simulink model "LDPC_sim"  (R2024a)
(part 16 of 20)

true;true;true;true;true;true;true;true;true;true;true;true;true;true;true;true;true;true;true;true;true;true;true;true;true;true;true;true;true;true;true;true;true;true;true;true;true;true;true;true;true;true;true;true;true;true;true;true;true;true;true;true;true;true;true;true;true;true;true;true;true;true;true;true;true;true;true;true;true;true;true;true;true;true;true;true;true;true;true;true;true;true;true;true;true;true;true;true;true;true;true;true;true;true;true;true;true;true;true;true;true;true;true;true;true;true;true;true;true;true;true;true;true;true;true;true;true;true;true;true;true;true;true;true;true;true;true;true;true;true;true;true;true;true;true;true;true;true;true;true;true;true;true;true;true;true;true;true;true;true;true;true;true;true;true;true;true;true;true;true;true;true;true;true;true;true;true;true;true;true;true;true;true;true;true;true;true;true;true;true;true;true;true;true;true;true;true;true;true;true;true;true;true;true;true;true;true;true;true;true;true;true;true;true;true;true;true;true;true;true;true;true;true;true;true;true;true;true;true;true;true;true;true;true;true;true;true;true;true;true;true;true;true;true;true;true;true;true;true;true;true;true;true;true;true;true;true;true;true;true;true;true;true;true;true;true;true;true;true;true;true;true;true;true;true;true;true;true;true;true;true;true;true;true;true;true;true;true;true;true;true;true;true;true;true;true;true;true;true;true;true;true;true;true;true;true;true;true;true;true;true;true;true;true;true;true;true;true;true;true;true;true;true;true;true;true;true;true;true;true;true;true;true;true;true;true;true;true;true;true;true;true;true;true;true;true;true;true;true;true;true;true;true;true;true;true;true;true;true;true;true;true;true;true;true;true;true;true;true;true;true;true;true;true;true;true;true;true;true;true;true;true;true;true;true;true;true;true;true;true;true;true;true;true;true;true;true;true;true;true;true;true;true;true;true;true;true;true;true;true;true;true;true;true;true;true;true;true;true;true;true;true;true;true;true;true;true;true;true;true;true;true;true;true;true;true;true;true;true;true;true;true;true;true;true;true;true;true;true;true;true;true;true;true;true;true;true;true;true;true;true;true;true;true;true;true;true;true;true;true;true;true;true;true;true;true;true;true;true;true;true;true;true;true;true;true;true;true;true;true;true;true;true;true;true;true;true;true;true;true;true;true;true;true;true;true;true;true;true;true;true;true;true;true;true;true;true;true;true;true;true;true;true;true;true;true;true;true;true;true;true;true;true;true;true;true;true;true;true;true;true;true;true;true;true;true;true;true;true;true;true;true;true;true;true;true;true;true;true;true;true;true;true;true;true;true;true;true;true;true;true;true;true;true;true;true;true;true;true;true;true;true;true;true;true;true;true;true;true;true;true;true;true;true;true;true;true;true;true;true;true;true;true;true;true;true;true;true;true;true;true;true;true;true;true;true;true;true;true;true;true;true;true;true;true;true;true;true;true;true;true;true;true;true;true;true;true;true;true;true;true;true;true;true;true;true;true;true;true;true;true;true;true;true;true;true;true;true;true;true;true;true;true;true;true;true;true;true;true;true;true;true;true;true;true;true;true;true;true;true;true;true;true;true;true;true;true;true;true;true;true;true;true;true;true;true;true;true;true;true;true;true;true;true;true;true;true;true;true;true;true;true;true;true;true;true;true;true;true;true;true;true;true;true;true;true;true;true;true;true;true;true;true;true;true;true;true;true;true;true;true;true;true;true;true;true;true;true;true;true;true;true;true;true;true;true;true;true;true;true;true;true;true;true;true;true;true;true;true;true;true;true;true;true;true;true;true;true;true;true;true;true;true;true;true;true;true;true;true;true;true;true;true;true;true;true;true;true;true;true;true;true;true;true;true;true;true;true;true;true;true;true;true;true;true;true;true;true;true;true;true;true;true;true;true;true;true;true;true;true;true;true;true;true;true;true;true;true;true;true;true;true;true;true;true;true;true;true;true;true;true;true;true;true;true;true;true;true;true;true;true;true;true;true;true;true;true;true;true;true;true;true;true;true;true;true;true;true;true;true;true;true;true;true;true;true;true;true;true;true;true;true;true;true;true;true;true;true;true;true;true;true;true;true;true;true;true;true;true;true;true;true;true;true;true;true;true;true;true;true;true;true;true;true;true;true;true;true;true;true;true;true;true;true;true;true;true;true;true;true;true;true;true;true;true;true;true;true;true;true;true;true;true;true;true;true;true;true;true;true;true;true;true;true;true;true;true;true;true;true;true;true;true;true;true;true;true;true;true;true;true;true;true;true;true;true;true;true;true;true;true;true;true;true;true;true;true;true;true;true;true;true;true;true;true;true;true;true;true;true;true;true;true;true;true;true;true;true;true;true;true;true;true;true;true;true;true;true;true;true;true;true;true;true;true;true;true;true;true;true;true;true;true;true;true;true;true;true;true;true;true;true;true;true;true;true;true;true;true;true;true;true;true;true;true;true;true;true;true;true;true;true;true;true;true;true;true;true;true;true;true;true;true;true;true;true;true;true;true;true;true;true;true;true;true;true;true;true;true;true;true;true;true;true;true;true;true;true;true;true;true;true;true;true;true;true;true;true;true;true;true;true;true;true;true;true;true;true;true;true;true;true;true;true;true;true;true;true;true;true;true;true;true;true;true;true;true;true;true;true;true;true;true;true;true;true;true;true;true;true;true;true;true;true;true;true;true;true;true;true;true;true;true;true;true;true;true;true;true;true;true;true;true;true;true;true;true;true;true;true;true;true;true;true;true;true;true;true;true;true;true;true;true;true;true;true;true;true;true;true;true;true;true;true;true;true;true;true;true;true;true;true;true;true;true;true;true;true;true;true;true;true;true;true;true;true;true;true;true;true;true;true;true;true;true;true;true;true;true;true;true;true;true;true;true;true;true;true;true;true;true;true;true;true;true;true;true;true;true;true;true;true;true;true;true;true;true;true;true;true;true;true;true;true;true;true;true;true;true;true;true;true;true;true;true;true;true;true;true;true;true;true;true;true;true;true;true;true;true;true;true;true;true;true;true;true;true;true;true;true;true;true;true;true;true;true;true;true;true;true;true;true;true;true;true;true;true;true;true;true;true;true;true;true;true;true;true;true;true;true;true;true;true;true;true;true;true;true;true;true;true;true;true;true;true;true;true;true;true;true;true;true;true;true;true;true;true;true;true;true;true;true;true;true;true;true;true;true;true;true;true;true;true;true;true;true;true;true;true;true;true;true;true;true;true;true;true;true;true;true;true;true;true;true;true;true;true;true;true;true;true;true;true;true;true;true;true;true;true;true;true;true;true;true;true;true;true;true;true;true;true;true;true;true;true;true;true;true;true;true;true;true;true;true;true;true;true;true;true;true;true;true;true;true;true;true;true;true;true;true;true;true;true;true;true;true;true;true;true;true;true;true;true;true;true;true;true;true;true;true;true;true;true;true;true;true;true;true;true;true;true;true;true;true;true;true;true;true;true;true;true;true;true;true;true;true;true;true;true;true;true;true;true;true;true;true;true;true;true;true;true;true;true;true;true;true;true;true;true;true;true;true;true;true;true;true;true;true;true;true;true;true;true;true;true;true;true;true;true;true;true;true;true;true;true;true;true;true;true;true;true;true;true;true;true;true;true;true;true;true;true;true;true;true;true;true;true;true;true;true;true;true;true;true;true;true;true;true;true;true;true;true;true;true;true;true;true;true;true;true;true;true;true;true;true;true;true;true;true;true;true;true;true;true;true;true;true;true;true;true;true;true;true;true;true;true;true;true;true;true;true;true;true;true;true;true;true;true;true;true;true;true;true;true;true;true;true;true;true;true;true;true;true;true;true;true;true;true;true;true;true;true;true;true;true;true;true;true;true;true;true;true;true;true;true;true;true;true;true;true;true;true;true;true;true;true;true;true;true;true;true;true;true;true;true;true;true;true;true;true;true;true;true;true;true;true;true;true;true;true;true;true;true;true;true;true;true;true;true;true;true;true;true;true;true;true;true;true;true;true;true;true;true;true;true;true;true;true;true;true;true;true;true;true;true;true;true;true;true;true;true;true;true;true;true;true;true;true;true;true;true;true;true;true;true;true;true;true;true;true;true;true;true;true;true;true;true;true;true;true;true;true;true;true;true;true;true;true;true;true;true;true;true;true;true;true;true;true;true;true;true;true;true;true;true;true;true;true;true;true;true;true;true;true;true;true;true;true;true;true;true;true;true;true;true;true;true;true;true;true;true;true;true;true;true;true;true;true;true;true;true;true;true;true;true;true;true;true;true;true;true;true;true;true;true;true;true;true;true;true;true;true;true;true;true;true;true;true;true;true;true;true;true;true;true;true;true;true;true;true;true;true;true;true;true;true;true;true;true;true;true;true;true;true;true;true;true;true;true;true;true;true;true;true;true;true;true;true;true;true;true;true;true;true;true;true;true;true;true;true;true;true;true;true;true;true;true;true;true;true;true;true;true;true;true;true;true;true;true;true;true;true;true;true;true;true;true;true;true;true;true;true;true;true;true;true;true;true;true;true;true;true;true;true;true;true;true;true;true;true;true;true;true;true;true;true;true;true;true;true;true;true;true;true;true;true;true;true;true;true;true;true;true;true;true;true;true;true;true;true;true;true;true;true;true;true;true;true;true;true;true;true;true;true;true;true;true;true;true;true;true;true;true;true;true;true;true;true;true;true;true;true;true;true;true;true;true;true;true;true;true;true;true;true;true;true;true;true;true;true;true;true;true;true;true;true;true;true;true;true;true;true;true;true;true;true;true;true;true;true;true;true;true;true;true;true;true;true;true;true;true;true;true;true;true;true;true;true;true;true;true;true;true;true;true;true;true;true;true;true;true;true;true;true;true;true;true;true;true;true;true;true;true;true;true;true;true;true;true;true;true;true;true;true;true;true;true;true;true;true;true;true;true;true;true;true;true;true;true;true;true;true;true;true;true;true;true;true;true;true;true;true;true;true;true;true;true;true;true;true;true;true;true;true;true;true;true;true;true;true;true;true;true;true;true;true;true;true;true;true;true;true;true;true;true;true;true;true;true;true;true;true;true;true;true;true;true;true;true;true;true;true;true;true;true;true;true;true;true;true;true;true;true;true;true;true;true;true;true;true;true;true;true;true;true;true;true;true;true;true;true;true;true;true;true;true;true;true;true;true;true;true;true;true;true;true;true;true;true;true;true;true;true;true;true;true;true;true;true;true;true;true;true;true;true;true;true;true;true;true;true;true;true;true;true;true;true;true;true;true;true;true;true;true;true;true;true;true;true;true;true;true;true;true;true;true;true;true;true;true;true;true;true;true;true;true;true;true;true;true;true;true;true;true;true;true;true;true;true;true;true;true;true;true;true;true;true;true;true;true;true;true;true;true;true;true;true;true;true;true;true;true;true;true;true;true;true;true;true;true;true;true;true;true;true;true;true;true;true;true;true;true;true;true;true;true;true;true;true;true;true;true;true;true;true;true;true;true;true;true;true;true;true;true;true;true;true;true;true;true;true;true;true;true;true;true;true;true;true;true;true;true;true;true;true;true;true;true;true;true;true;true;true;true;true;true;true;true;true;true;true;true;true;true;true;true;true;true;true;true;true;true;true;true;true;true;true;true;true;true;true;true;true;true;true;true;true;true;true;true;true;true;true;true;true;true;true;true;true;true;true;true;true;true;true;true;true;true;true;true;true;true;true;true;true;true;true;true;true;true;true;true;true;true;true;true;true;true;true;true;true;true;true;true;true;true;true;true;true;true;true;true;true;true;true;true;true;true;true;true;true;true;true;true;true;true;true;true;true;true;true;true;true;true;true;true;true;true;true;true;true;true;true;true;true;true;true;true;true;true;true;true;true;true;true;true;true;true;true;true;true;true;true;true;true;true;true;true;true;true;true;true;true;true;true;true;true;true;true;true;true;true;true;true;true;true;true;true;true;true;true;true;true;true;true;true;true;true;true;true;true;true;true;true;true;true;true;true;true;true;true;true;true;true;true;true;true;true;true;true;true;true;true;true;true;true;true;true;true;true;true;true;true;true;true;true;true;true;true;true;true;true;true;true;true;true;true;true;true;true;true;true;true;true;true;true;true;true;true;true;true;true;true;true;true;true;true;true;true;true;true;true;true;true;true;true;true;true;true;true;true;true;true;true;true;true;true;true;true;true;true;true;true;true;true;true;true;true;true;true;true;true;true;true;true;true;true;true;true;true;true;true;true;true;true;true;true;true;true;true;true;true;true;true;true;true;true;true;true;true;true;true;true;true;true;true;true;true;true;true;true;true;true;true;true;true;true;true;true;true;true;true;true;true;true;true;true;true;true;true;true;true;true;true;true;true;true;true;true;true;true;true;true;true;true;true;true;true;true;true;true;true;true;true;true;true;true;true;true;true;true;true;true;true;true;true;true;true;true;true;true;true;true;true;true;true;true;true;true;true;true;true;true;true;true;true;true;true;true;true;true;true;true;true;true;true;true;true;true;true;true;true;true;true;true;true;true;true;true;true;true;true;true;true;true;true;true;true;true;true;true;true;true;true;true;true;true;true;true;true;true;true;true;true;true;true;true;true;true;true;true;true;true;true;true;true;true;true;true;true;true;true;true;true;true;true;true;true;true;true;true;true;true;true;true;true;true;true;true;true;true;true;true;true;true;true;true;true;true;true;true;true;true;true;true;true;true;true;true;true;true;true;true;true;true;true;true;true;true;true;true;true;true;true;true;true;true;true;true;true;true;true;true;true;true;true;true;true;true;true;true;true;true;true;true;true;true;true;true;true;true;true;true;true;true;true;true;true;true;true;true;true;true;true;true;true;true;true;true;true;true;true;true;true;true;true;true;true;true;true;true;true;true;true;true;true;true;true;true;true;true;true;true;true;true;true;true;true;true;true;true;true;true;true;true;true;true;true;true;true;true;true;true;true;true;true;true;true;true;true;true;true;true;true;true;true;true;true;true;true;true;true;true;true;true;true;true;true;true;true;true;true;true;true;true;true;true;true;true;true;true;true;true;true;true;true;true;true;true;true;true;true;true;true;true;true;true;true;true;true;true;true;true;true;true;true;true;true;true;true;true;true;true;true;true;true;true;true;true;true;true;true;true;true;true;true;true;true;true;true;true;true;true;true;true;true;true;true;true;true;true;true;true;true;true;true;true;true;true;true;true;true;true;true;true;true;true;true;true;true;true;true;true;true;true;true;true;true;true;true;true;true;true;true;true;true;true;true;true;true;true;true;true;true;true;true;true;true;true;true;true;true;true;true;true;true;true;true;true;true;true;true;true;true;true;true;true;true;true;true;true;true;true;true;true;true;true;true;true;true;true;true;true;true;true;true;true;true;true;true;true;true;true;true;true;true;true;true;true;true;true;true;true;true;true;true;true;true;true;true;true;true;true;true;true;true;true;true;true;true;true;true;true;true;true;true;true;true;true;true;true;true;true;true;true;true;true;true;true;true;true;true;true;true;true;true;true;true;true;true;true;true;true;true;true;true;true;true;true;true;true;true;true;true;true;true;true;true;true;true;true;true;true;true;true;true;true;true;true;true;true;true;true;true;true;true;true;true;true;true;true;true;true;true;true;true;true;true;true;true;true;true;true;true;true;true;true;true;true;true;true;true;true;true;true;true;true;true;true;true;true;true;true;true;true;true;true;true;true;true;true;true;true;true;true;true;true;true;true;true;true;true;true;true;true;true;true;true;true;true;true;true;true;true;true;true;true;true;true;true;true;true;true;true;true;true;true;true;true;true;true;true;true;true;true;true;true;true;true;true;true;true;true;true;true;true;true;true;true;true;true;true;true;true;true;true;true;true;true;true;true;true;true;true;true;true;true;true;true;true;true;true;true;true;true;true;true;true;true;true;true;true;true;true;true;true;true;true;true;true;true;true;true;true;true;true;true;true;true;true;true;true;true;true;true;true;true;true;true;true;true;true;true;true;true;true;true;true;true;true;true;true;true;true;true;true;true;true;true;true;true;true;true;true;true;true;true;true;true;true;true;true;true;true;true;true;true;true;true;true;true;true;true;true;true;true;true;true;true;true;true;true;true;true;true;true;true;true;true;true;true;true;true;true;true;true;true;true;true;true;true;true;true;true;true;true;true;true;true;true;true;true;true;true;true;true;true;true;true;true;true;true;true;true;true;true;true;true;true;true;true;true;true;true;true;true;true;true;true;true;true;true;true;true;true;true;true;true;true;true;true;true;true;true;true;true;true;true;true;true;true;true;true;true;true;true;true;true;true;true;true;true;true;true;true;true;true;true;true;true;true;true;true;true;true;true;true;true;true;true;true;true;true;true;true;true;true;true;true;true;true;true;true;true;true;true;true;true;true;true;true;true;true;true;true;true;true;true;true;true;true;true;true;true;true;true;true;true;true;true;true;true;true;true;true;true;true;true;true;true;true;true;true;true;true;true;true;true;true;true;true;true;true;true;true;true;true;true;true;true;true;true;true;true;true;true;true;true;true;true;true;true;true;true;true;true;true;true;true;true;true;true;true;true;true;true;true;true;true;true;true;true;true;true;true;true;true;true;true;true;true;true;true;true;true;true;true;true;true;true;true;true;true;true;true;true;true;true;true;true;true;true;true;true;true;true;true;true;true;true;true;true;true;true;true;true;true;true;true;true;true;true;true;true;true;true;true;true;true;true;true;true;true;true;true;true;true;true;true;true;true;true;true;true;true;true;true;true;true;true;true;true;true;true;true;true;true;true;true;true;true;true;true;true;true;true;true;true;true;true;true;true;true;true;true;true;true;true;true;true;true;true;true;true;true;true;true;true;true;true;true;true;true;true;true;true;true;true;true;true;true;true;true;true;true;true;true;true;true;true;true;true;true;true;true;true;true;true;true;true;true;true;true;true;true;true;true;true;true;true;true;true;true;true;true;true;true;true;true;true;true;true;true;true;true;true;true;true;true;true;true;true;true;true;true;true;true;true;true;true;true;true;true;true;true;true;true;true;true;true;true;true;true;true;true;true;true;true;true;true;true;true;true;true;true;true;true;true;true;true;true;true;true;true;true;true;true;true;true;true;true;true;true;true;true;true;true;true;true;true;true;true;true;true;true;true;true;true;true;true;true;true;true;true;true;true;true;true;true;true;true;true;true;true;true;true;true;true;true;true;true;true;true;true;true;true;true;true;true;true;true;true;true;true;true;true;true;true;true;true;true;true;true;true;true;true;true;true;true;true;true;true;true;true;true;true;true;true;true;true;true;true;true;true;true;true;true;true;true;true;true;true;true;true;true;true;true;true;true;true;true;true;true;true;true;true;true;true;true;true;true;true;true;true;true;true;true;true;true;true;true;true;true;true;true;true;true;true;true;true;true;true;true;true;true;true;true;true;true;true;true;true;true;true;true;true;true;true;true;true;true;true;true;true;true;true;true;true;true;true;true;true;true;true;true;true;true;true;true;true;true;true;true;true;true;true;true;true;true;true;true;true;true;true;true;true;true;true;true;true;true;true;true;true;true;true;true;true;true;true;true;true;true;true;true;true;true;true;true;true;true;true;true;true;true;true;true;true;true;true;true;true;true;true;true;true;true;true;true;true;true;true;true;true;true;true;true;true;true;true;true;true;true;true;true;true;true;true;true;true;true;true;true;true;true;true;true;true;true;true;true;true;true;true;true;true;true;true;true;true;true;true;true;true;true;true;true;true;true;true;true;true;true;true;true;true;true;true;true;true;true;true;true;true;true;true;true;true;true;true;true;true;true;true;true;true;true;true;true;true;true;true;true;true;true;true;true;true;true;true;true;true;true;true;true;true;true;true;true;true;true;true;true;true;true;true;true;true;true;true;true;true;true;true;true;true;true;true;true;true;true;true;true;true;true;true;true;true;true;true;true;true;true;true;true;true;true;true;true;true;true;true;true;true;true;true;true;true;true;true;true;true;true;true;true;true;true;true;true;true;true;true;true;true;true;true;true;true;true;true;true;true;true;true;true;true;true;true;true;true;true;true;true;true;true;true;true;true;true;true;true;true;true;true;true;true;true;true;true;true;true;true;true;true;true;true;true;true;true;true;true;true;true;true;true;true;true;true;true;true;true;true;true;true;true;true;true;true;true;true;true;true;true;true;true;true;true;true;true;true;true;true;true;true;true;true;true;true;true;true;true;true;true;true;true;true;true;true;true;true;true;true;true;true;true;true;true;true;true;true;true;true;true;true;true;true;true;true;true;true;true;true;true;true;true;true;true;true;true;true;true;true;true;true;true;true;true;true;true;true;true;true;true;true;true;true;true;true;true;true;true;true;true;true;true;true;true;true;true;true;true;true;true;true;true;true;true;true;true;true;true;true;true;true;true;true;true;true;true;true;true;true;true;true;true;true;true;true;true;true;true;true;true;true;true;true;true;true;true;true;true;true;true;true;true;true;true;true;true;true;true;true;true;true;true;true;true;true;true;true;true;true;true;true;true;true;true;true;true;true;true;true;true;true;true;true;true;true;true;true;true;true;true;true;true;true;true;true;true;true;true;true;true;true;true;true;true;true;true;true;true;true;true;true;true;true;true;true;true;true;true;true;true;true;true;true;true;true;true;true;true;true;true;true;true;true;true;true;true;true;true;true;true;true;true;true;true;true;true;true;true;true;true;true;true;true;true;true;true;true;true;true;true;true;true;true;true;true;true;true;true;true;true;true;true;true;true;true;true;true;true;true;true;true;true;true;true;true;true;true;true;true;true;true;true;true;true;true;true;true;true;true;true;true;true;true;true;true;true;true;true;true;true;true;true;true;true;true;true;true;true;true;true;true;true;true;true;true;true;true;true;true;true;true;true;true;true;true;true;true;true;true;true;true;true;true;true;true;true;true;true;true;true;true;true;true;true;true;true;true;true;true;true;true;true;true;true;true;true;true;true;true;true;true;true;true;true;true;true;true;true;true;true;true;true;true;true;true;true;true;true;true;true;true;true;true;true;true;true;true;true;true;true;true;true;true;true;true;true;true;true;true;true;true;true;true;true;true;true;true;true;true;true;true;true;true;true;true;true;true;true;true;true;true;true;true;true;true;true;true;true;true;true;true;true;true;true;true;true;true;true;true;true;true;true;true;true;true;true;true;true;true;true;true;true;true;true;true;true;true;true;true;true;true;true;true;true;true;true;true;true;true;true;true;true;true;true;true;true;true;true;true;true;true;true;true;true;true;true;true;true;true;true;true;true;true;true;true;true;true;true;true;true;true;true;true;true;true;true;true;true;true;true;true;true;true;true;true;true;true;true;true;true;true;true;true;true;true;true;true;true;true;true;true;true;true;true;true;true;true;true;true;true;true;true;true;true;true;true;true;true;true;true;true;true;true;true;true;true;true;true;true;true;true;true;true;true;true;true;true;true;true;true;true;true;true;true;true;true;true;true;true;true;true;true;true;true;true;true;true;true;true;true;true;true;true;true;true;true;true;true;true;true;true;true;true;true;true;true;true;true;true;true;true;true;true;true;true;true;true;true;true;true;true;true;true;true;true;true;true;true;true;true;true;true;true;true;true;true;true;true;true;true;true;true;true;true;true;true;true;true;true;true;true;true;true;true;true;true;true;true;true;true;true;true;true;true;true;true;true;true;true;true;true;true;true;true;true;true;true;true;true;true;true;true;true;true;true;true;true;true;true;true;true;true;true;true;true;true;true;true;true;true;true;true;true;true;true;true;true;true;true;true;true;true;true;true;true;true;true;true;true;true;true;true;true;true;true;true;true;true;true;true;true;true;true;true;true;true;true;true;true;true;true;true;true;true;true;true;true;true;true;true;true;true;true;true;true;true;true;true;true;true;true;true;true;true;true;true;true;true;true;true;true;true;true;true;true;true;true;true;true;true;true;true;true;true;true;true;true;true;true;true;true;true;true;true;true;true;true;true;true;true;true;true;true;true;true;true;true;true;true;true;true;true;true;true;true;true;true;true;true;true;true;true;true;true;true;true;true;true;true;true;true;true;true;true;true;true;true;true;true;true;true;true;true;true;true;true;true;true;true;true;true;true;true;true;true;true;true;true;true;true;true;true;true;true;true;true;true;true;true;true;true;true;true;true;true;true;true;true;true;true;true;true;true;true;true;true;true;true;true;true;true;true;true;true;true;true;true;true;true;true;true;true;true;true;true;true;true;true;true;true;true;true;true;true;true;true;true;true;true;true;true;true;true;true;true;true;true;true;true;true;true;true;true;true;true;true;true;true;true;true;true;true;true;true;true;true;true;true;true;true;true;true;true;true;true;true;true;true;true;true;true;true;true;true;true;true;true;true;true;true;true;true;true;true;true;true;true;true;true;true;true;true;true;true;true;true;true;true;true;true;true;true;true;true;true;true;true;true;true;true;true;true;true;true;true;true;true;true;true;true;true;true;true;true;true;true;true;true;true;true;true;true;true;true;true;true;true;true;true;true;true;true;true;true;true;true;true;true;true;true;true;true;true;true;true;true;true;true;true;true;true;true;true;true;true;true;true;true;true;true;true;true;true;true;true;true;true;true;true;true;true;true;true;true;true;true;true;true;true;true;true;true;true;true;true;true;true;true;true;true;true;true;true;true;true;true;true;true;true;true;true;true;true;true;true;true;true;true;true;true;true;true;true;true;true;true;true;true;true;true;true;true;true;true;true;true;true;true;true;true;true;true;true;true;true;true;true;true;true;true;true;true;true;true;true;true;true;true;true;true;true;true;true;true;true;true;true;true;true;true;true;true;true;true;true;true;true;true;true;true;true;true;true;true;true;true;true;true;true;true;true;true;true;true;true;true;true;true;true;true;true;true;true;true;true;true;true;true;true;true;true;true;true;true;true;true;true;true;true;true;true;true;true;true;true;true;true;true;true;true;true;true;true;true;true;true;true;true;true;true;true;true;true;true;true;true;true;true;true;true;true;true;true;true;true;true;true;true;true;true;true;true;true;true;true;true;true;true;true;true;true;true;true;true;true;true;true;true;true;true;true;true;true;true;true;true;true;true;true;true;true;true;true;true;true;true;true;true;true;true;true;true;true;true;true;true;true;true;true;true;true;true;true;true;true;true;true;true;true;true;true;true;true;true;true;true;true;true;true;true;true;true;true;true;true;true;true;true;true;true;true;true;true;true;true;true;true;true;true;true;true;true;true;true;true;true;true;true;true;true;true;true;true;true;true;true;true;true;true;true;true;true;true;true;true;true;true;true;true;true;true;true;true;true;true;true;true;true;true;true;true;true;true;true;true;true;true;true;true;true;true;true;true;true;true;true;true;true;true;true;true;true;true;true;true;true;true;true;true;true;true;true;true;true;true;true;true;true;true;true;true;true;true;true;true;true;true;true;true;true;true;true;true;true;true;true;true;true;true;true;true;true;true;true;true;true;true;true;true;true;true;true;true;true;true;true;true;true;true;true;true;true;true;true;true;true;true;true;true;true;true;true;true;true;true;true;true;true;true;true;true;true;true;true;true;true;true;true;true;true;true;true;true;true;true;true;true;true;true;true;true;true;true;true;true;true;true;true;true;true;true;true;true;true;true;true;true;true;true;true;true;true;true;true;true;true;true;true;true;true;true;true;true;true;true;true;true;true;true;true;true;true;true;true;true;true;true;true;true;true;true;true;true;true;true;true;true;true;true;true;true;true;true;true;true;true;true;true;true;true;true;true;true;true;true;true;true;true;true;true;true;true;true;true;true;true;true;true;true;true;true;true;true;true;true;true;true;true;true;true;true;true;true;true;true;true;true;true;true;true;true;true;true;true;true;true;true;true;true;true;true;true;true;true;true;true;true;true;true;true;true;true;true;true;true;true;true;true;true;true;true;true;true;true;true;true;true;true;true;true;true;true;true;true;true;true;true;true;true;true;true;true;true;true;true;true;true;true;true;true;true;true;true;true;true;true;true;true;true;true;true;true;true;true;true;true;true;true;true;true;true;true;true;true;true;true;true;true;true;true;true;true;true;true;true;true;true;true;true;true;true;true;true;true;true;true;true;true;true;true;true;true;true;true;true;true;true;true;true;true;true;true;true;true;true;true;true;true;true;true;true;true;true;true;true;true;true;true;true;true;true;true;true;true;true;true;true;true;true;true;true;true;true;true;true;true;true;true;true;true;true;true;true;true;true;true;true;true;true;true;true;true;true;true;true;true;true;true;true;true;true;true;true;true;true;true;true;true;true;true;true;true;true;true;true;true;true;true;true;true;true;true;true;true;true;true;true;true;true;true;true;true;true;true;true;true;true;true;true;true;true;true;true;true;true;true;true;true;true;true;true;true;true;true;true;true;true;true;true;true;true;true;true;true;true;true;true;true;true;true;true;true;true;true;true;true;true;true;true;true;true;true;true;true;true;true;true;true;true;true;true;true;true;true;true;true;true;true;true;true;true;true;true;true;true;true;true;true;true;true;true;true;true;true;true;true;true;true;true;true;true;true;true;true;true;true;true;true;true;true;true;true;true;true;true;true;true;true;true;true;true;true;true;true;true;true;true;true;true;true;true;true;true;true;true;true;true;true;true;true;true;true;true;true;true;true;true;true;true;true;true;true;true;true;true;true;true;true;true;true;true;true;true;true;true;true;true;true;true;true;true;true;true;true;true;true;true;true;true;true;true;true;true;true;true;true;true;true;true;true;true;true;true;true;true;true;true;true;true;true;true;true;true;true;true;true;true;true;true;true;true;true;true;true;true;true;true;true;true;true;true;true;true;true;true;true;true;true;true;true;true;true;true;true;true;true;true;true;true;true;true;true;true;true;true;true;true;true;true;true;true;true;true;true;true;true;true;true;true;true;true;true;true;true;true;true;true;true;true;true;true;true;true;true;true;true;true;true;true;true;true;true;true;true;true;true;true;true;true;true;true;true;true;true;true;true;true;true;true;true;true;true;true;true;true;true;true;true;true;true;true;true;true;true;true;true;true;true;true;true;true;true;true;true;true;true;true;true;true;true;true;true;true;true;true;true;true;true;true;true;true;true;true;true;true;true;true;true;true;true;true;true;true;true;true;true;true;true;true;true;true;true;true;true;true;true;true;true;true;true;true;true;true;true;true;true;true;true;true;true;true;true;true;true;true;true;true;true;true;true;true;true;true;true;true;true;true;true;true;true;true;true;true;true;true;true;true;true;true;true;true;true;true;true;true;true;true;true;true;true;true;true;true;true;true;true;true;true;true;true;true;true;true;true;true;true;true;true;true;true;true;true;true;true;true;true;true;true;true;true;true;true;true;true;true;true;true;true;true;true;true;true;true;true;true;true;true;true;true;true;true;true;true;true;true;true;true;true;true;true;true;true;true;true;true;true;true;true;true;true;true;true;true;true;true;true;true;true;true;true;true;true;true;true;true;true;true;true;true;true;true;true;true;true;true;true;true;true;true;true;true;true;true;true;true;true;true;true;true;true;true;true;true;true;true;true;true;true;true;true;true;true;true;true;true;true;true;true;true;true;true;true;true;true;true;true;true;true;true;true;true;true;true;true;true;true;true;true;true;true;true;true;true;true;true;true;true;true;true;true;true;true;true;true;true;true;true;true;true;true;true;true;true;true;true;true;true;true;true;true;true;true;true;true;true;true;true;true;true;true;true;true;true;true;true;true;true;true;true;true;true;true;true;true;true;true;true;true;true;true;true;true;true;true;true;true;true;true;true;true;true;true;true;true;true;true;true;true;true;true;true;true;true;true;true;true;true;true;true;true;true;true;true;true;true;true;true;true;true;true;true;true;true;true;true;true;true;true;true;true;true;true;true;true;true;true;true;true;true;true;true;true;true;true;true;true;true;true;true;true;true;true;true;true;true;true;true;true;true;true;true;true;true;true;true;true;true;true;true;true;true;true;true;true;true;true;true;true;true;true;true;true;true;true;true;true;true;true;true;true;true;true;true;true;true;true;true;true;true;true;true;true;true;true;true;true;true;true;true;true;true;true;true;true;true;true;true;true;true;true;true;true;true;true;true;true;true;true;true;true;true;true;true;true;true;true;true;true;true;true;true;true;true;true;true;true;true;true;true;true;true;true;true;true;true;true;true;true;true;true;true;true;true;true;true;true;true;true;true;true;true;true;true;true;true;true;true;true;true;true;true;true;true;true;true;true;true;true;true;true;true;true;true;true;true;true;true;true;true;true;true;true;true;true;true;true;true;true;true;true;true;true;true;true;true;true;true;true;true;true;true;true;true;true;true;true;true;true;true;true;true;true;true;true;true;true;true;true;true;true;true;true;true;true;true;true;true;true;true;true;true;true;true;true;true;true;true;true;true;true;true;true;true;true;true;true;true;true;true;true;true;true;true;true;true;true;true;true;true;true;true;true;true;true;true;true;true;true;true;true;true;true;true;true;true;true;true;true;true;true;true;true;true;true;true;true;true;true;true;true;true;true;true;true;true;true;true;true;true;true;true;true;true;true;true;true;true;true;true;true;true;true;true;true;true;true;true;true;true;true;true;true;true;true;true;true;true;true;true;true;true;true;true;true;true;true;true;true;true;true;true;true;true;true;true;true;true;true;true;true;true;true;true;true;true;true;true;true;true;true;true;true;true;true;true;true;true;true;true;true;true;true;true;true;true;true;true;true;true;true;true;true;true;true;true;true;true;true;true;true;true;true;true;true;true;true;true;true;true;true;true;true;true;true;true;true;true;true;true;true;true;true;true;true;true;true;true;true;true;true;true;true;true;true;true;true;true;true;true;true;true;true;true;true;true;true;true;true;true;true;true;true;true;true;true;true;true;true;true;true;true;true;true;true;true;true;true;true;true;true;true;true;true;true;true;true;true;true;true;true;true;true;true;true;true;true;true;true;true;true;true;true;true;true;true;true;true;true;true;true;true;true;true;true;true;true;true;true;true;true;true;true;true;true;true;true;true;true;true;true;true;true;true;true;true;true;true;true;true;true;true;true;true;true;true;true;true;true;true;true;true;true;true;true;true;true;true;true;true;true;true;true;true;true;true;true;true;true;true;true;true;true;true;true;true;true;true;true;true;true;true;true;true;true;true;true;true;true;true;true;true;true;true;true;true;true;true;true;true;true;true;true;true;true;true;true;true;true;true;true;true;true;true;true;true;true;true;true;true;true;true;true;true;true;true;true;true;true;true;true;true;true;true;true;true;true;true;true;true;true;true;true;true;true;true;true;true;true;true;true;true;true;true;true;true;true;true;true;true;true;true;true;true;true;true;true;true;true;true;true;true;true;true;true;true;true;true;true;true;true;true;true;true;true;true;true;true;true;true;true;true;true;true;true;true;true;true;true;true;true;true;true;true;true;true;true;true;true;true;true;true;true;true;true;true;true;true;true;true;true;true;true;true;true;true;true;true;true;true;true;true;true;true;true;true;true;true;true;true;true;true;true;true;true;true;true;true;true;true;true;true;true;true;true;true;true;true;true;true;true;true;true;true;true;true;true;true;true;true;true;true;true;true;true;true;true;true;true;true;true;true;true;true;true;true;true;true;true;true;true;true;true;true;true;true;true;true;true;true;true;true;true;true;true;true;true;true;true;true;true;true;true;true;true;true;true;true;true;true;true;true;true;true;true;true;true;true;true;true;true;true;true;true;true;true;true;true;true;true;true;true;true;true;true;true;true;true;true;true;true;true;true;true;true;true;true;true;true;true;true;true;true;true;true;true;true;true;true;true;true;true;true;true;true;true;true;true;true;true;true;true;true;true;true;true;true;true;true;true;true;true;true;true;true;true;true;true;true;true;true;true;true;true;true;true;true;true;true;true;true;true;true;true;true;true;true;true;true;true;true;true;true;true;true;true;true;true;true;true;true;true;true;true;true;true;true;true;true;true;true;true;true;true;true;true;true;true;true;true;true;true;true;true;true;true;true;true;true;true;true;true;true;true;true;true;true;true;true;true;true;true;true;true;true;true;true;true;true;true;true;true;true;true;true;true;true;true;true;true;true;true;true;true;true;true;true;true;true;true;true;true;true;true;true;true;true;true;true;true;true;true;true;true;true;true;true;true;true;true;true;true;true;true;true;true;true;true;true;true;true;true;true;true;true;true;true;true;true;true;true;true;true;true;true;true;true;true;true;true;true;true;true;true;true;true;true;true;true;true;true;true;true;true;true;true;true;true;true;true;true;true;true;true;true;true;true;true;true;true;true;true;true;true;true;true;true;true;true;true;true;true;true;true;true;true;true;true;true;true;true;true;true;true;true;true;true;true;true;true;true;true;true;true;true;true;true;true;true;true;true;true;true;true;true;true;true;true;true;true;true;true;true;true;true;true;true;true;true;true;true;true;true;true;true;true;true;true;true;true;true;true;true;true;true;true;true;true;true;true;true;true;true;true;true;true;true;true;true;true;true;true;true;true;true;true;true;true;true;true;true;true;true;true;true;true;true;true;true;true;true;true;true;true;true;true;true;true;true;true;true;true;true;true;true;true;true;true;true;true;true;true;true;true;true;true;true;true;true;true;true;true;true;true;true;true;true;true;true;true;true;true;true;true;true;true;true;true;true;true;true;true;true;true;true;true;true;true;true;true;true;true;true;true;true;true;true;true;true;true;true;true;true;true;true;true;true;true;true;true;true;true;true;true;true;true;true;true;true;true;true;true;true;true;true;true;true;true;true;true;true;true;true;true;true;true;true;true;true;true;true;true;true;true;true;true;true;true;true;true;true;true;true;true;true;true;true;true;true;true;true;true;true;true;true;true;true;true;true;true;true;true;true;true;true;true;true;true;true;true;true;true;true;true;true;true;true;true;true;true;true;true;true;true;true;true;true;true;true;true;true;true;true;true;true;true;true;true;true;true;true;true;true;true;true;true;true;true;true;true;true;true;true;true;true;true;true;true;true;true;true;true;true;true;true;true;true;true;true;true;true;true;true;true;true;true;true;true;true;true;true;true;true;true;true;true;true;true;true;true;true;true;true;true;true;true;true;true;true;true;true;true;true;true;true;true;true;true;true;true;true;true;true;true;true;true;true;true;true;true;true;true;true;true;true;true;true;true;true;true;true;true;true;true;true;true;true;true;true;true;true;true;true;true;true;true;true;true;true;true;true;true;true;true;true;true;true;true;true;true;true;true;true;true;true;true;true;true;true;true;true;true;true;true;true;true;true;true;true;true;true;true;true;true;true;true;true;true;true;true;true;true;true;true;true;true;true;true;true;true;true;true;true;true;true;true;true;true;true;true;true;true;true;true;true;true;true;true;true;true;true;true;true;true;true;true;true;true;true;true;true;true;true;true;true;true;true;true;true;true;true;true;true;true;true;true;true;true;true;true;true;true;true;true;true;true;true;true;true;true;true;true;true;true;true;true;true;true;true;true;true;true;true;true;true;true;true;true;true;true;true;true;true;true;true;true;true;true;true;true;true;true;true;true;true;true;true;true;true;true;true;true;true;true;true;true;true;true;true;true;true;true;true;true;true;true;true;true;true;true;true;true;true;true;true;true;true;true;true;true;true;true;true;true;true;true;true;true;true;true;true;true;true;true;true;true;true;true;true;true;true;true;true;true;true;true;true;true;true;true;true;true;true;true;true;true;true;true;true;true;true;true;true;true;true;true;true;true;true;true;true;true;true;true;true;true;true;true;true;true;true;true;true;true;true;true;true;true;true;true;true;true;true;true;true;true;true;true;true;true;true;true;true;true;true;true;true;true;true;true;true;true;true;true;true;true;true;true;true;true;true;true;true;true;true;true;true;true;true;true;true;true;true;true;true;true;true;true;true;true;true;true;true;true;true;true;true;true;true;true;true;true;true;true;true;true;true;true;true;true;true;true;true;true;true;true;true;true;true;true;true;true;true;true;true;true;true;true;true;true;true;true;true;true;true;true;true;true;true;true;true;true;true;true;true;true;true;true;true;true;true;true;true;true;true;true;true;true;true;true;true;true;true;true;true;true;true;true;true;true;true;true;true;true;true;true;true;true;true;true;true;true;true;true;true;true;true;true;true;true;true;true;true;true;true;true;true;true;true;true;true;true;true;true;true;true;true;true;true;true;true;true;true;true;true;true;true;true;true;true;true;true;true;true;true;true;true;true;true;true;true;true;true;true;true;true;true;true;true;true;true;true;true;true;true;true;true;true;true;true;true;true;true;true;true;true;true;true;true;true;true;true;true;true;true;true;true;true;true;true;true;true;true;true;true;true;true;true;true;true;true;true;true;true;true;true;true;true;true;true;true;true;true;true;true;true;true;true;true;true;true;true;true;true;true;true;true;true;true;true;true;true;true;true;true;true;true;true;true;true;true;true;true;true;true;true;true;true;true;true;true;true;true;true;true;true;true;true;true;true;true;true;true;true;true;true;true;true;true;true;true;true;true;true;true;true;true;true;true;true;true;true;true;true;true;true;true;true;true;true;true;true;true;true;true;true;true;true;true;true;true;true;true;true;true;true;true;true;true;true;true;true;true;true;true;true;true;true;true;true;true;true;true;true;true;true;true;true;true;true;true;true;true;true;true;true;true;true;true;true;true;true;true;true;true;true;true;true;true;true;true;true;true;true;true;true;true;true;true;true;true;true;true;true;true;true;true;true;true;true;true;true;true;true;true;true;true;true;true;true;true;true;true;true;true;true;true;true;true;true;true;true;true;true;true;true;true;true;true;true;true;true;true;true;true;true;true;true;true;true;true;true;true;true;true;true;true;true;true;true;true;true;true;true;true;true;true;true;true;true;true;true;true;true;true;true;true;true;true;true;true;true;true;true;true;true;true;true;true;true;true;true;true;true;true;true;true;true;true;true;true;true;true;true;true;true;true;true;true;true;true;true;true;true;true;true;true;true;true;true;true;true;true;true;true;true;true;true;true;true;true;true;true;true;true;true;true;true;true;true;true;true;true;true;true;true;true;true;true;true;true;true;true;true;true;true;true;true;true;true;true;true;true;true;true;true;true;true;true;true;true;true;true;true;true;true;true;true;true;true;true;true;true;true;true;true;true;true;true;true;true;true;true;true;true;true;true;true;true;true;true;true;true;true;true;true;true;true;true;true;true;true;true;true;true;true;true;true;true;true;true;true;true;true;true;true;true;true;true;true;true;true;true;true;true;true;true;true;true;true;true;true;true;true;true;true;true;true;true;true;true;true;true;true;true;true;true;true;true;true;true;true;true;true;true;true;true;true;true;true;true;true;true;true;true;true;true;true;true;true;true;true;true;true;true;true;true;true;true;true;true;true;true;true;true;true;true;true;true;true;true;true;true;true;true;true;true;true;true;true;true;true;true;true;true;true;true;true;true;true;true;true;true;true;true;true;true;true;true;true;true;true;true;true;true;true;true;true;true;true;true;true;true;true;true;true;true;true;true;true;true;true;true;true;true;true;true;true;true;true;true;true;true;true;true;true;true;true;true;true;true;true;true;true;true;true;true;true;true;true;true;true;true;true;true;true;true;true;true;true;true;true;true;true;true;true;true;true;true;true;true;true;true;true;true;true;true;true;true;true;true;true;true;true;true;true;true;true;true;true;true;true;true;true;true;true;true;true;true;true;true;true;true;true;true;true;true;true;true;true;true;true;true;true;true;true;true;true;true;true;true;true;true;true;true;true;true;true;true;true;true;true;true;true;true;true;true;true;true;true;true;true;true;true;true;true;true;true;true;true;true;true;true;true;true;true;true;true;true;true;true;true;true;true;true;true;true;true;true;true;true;true;true;true;true;true;true;true;true;true;true;true;true;true;true;true;true;true;true;true;true;true;true;true;true;true;true;true;true;true;true;true;true;true;true;true;true;true;true;true;true;true;true;true;true;true;true;true;true;true;true;true;true;true;true;true;true;true;true;true;true;true;true;true;true;true;true;true;true;true;true;true;true;true;true;true;true;true;true;true;true;true;true;true;true;true;true;true;true;true;true;true;true;true;true;true;true;true;true;true;true;true;true;true;true;true;true;true;true;true;true;true;true;true;true;true;true;true;true;true;true;true;true;true;true;true;true;true;true;true;true;true;true;true;true;true;true;true;true;true;true;true;true;true;true;true;true;true;true;true;true;true;true;true;true;true;true;true;true;true;true;true;true;true;true;true;true;true;true;true;true;true;true;true;true;true;true;true;true;true;true;true;true;true;true;true;true;true;true;true;true;true;true;true;true;true;true;true;true;true;true;true;true;true;true;true;true;true;true;true;true;true;true;true;true;true;true;true;true;true;true;true;true;true;true;true;true;true;true;true;true;true;true;true;true;true;true;true;true;true;true;true;true;true;true;true;true;true;true;true;true;true;true;true;true;true;true;true;true;true;true;true;true;true;true;true;true;true;true;true;true;true;true;true;true;true;true;true;true;true;true;true;true;true;true;true;true;true;true;true;true;true;true;true;true;true;true;true;true;true;true;true;true;true;true;true;true;true;true;true;true;true;true;true;true;true;true;true;true;true;true;true;true;true;true;true;true;true;true;true;true;true;true;true;true;true;true;true;true;true;true;true;true;true;true;true;true;true;true;true;true;true;true;true;true;true;true;true;true;true;true;true;true;true;true;true;true;true;true;true;true;true;true;true;true;true;true;true;true;true;true;true;true;true;true;true;true;true;true;true;true;true;true;true;true;true;true;true;true;true;true;true;true;true;true;true;true;true;true;true;true;true;true;true;true;true;true;true;true;true;true;true;true;true;true;true;true;true;true;true;true;true;true;true;true;true;true;true;true;true;true;true;true;true;true;true;true;true;true;true;true;true;true;true;true;true;true;true;true;true;true;true;true;true;true;true;true;true;true;true;true;true;true;true;true;true;true;true;true;true;true;true;true;true;true;true;true;true;true;true;true;true;true;true;true;true;true;true;true;true;true;true;true;true;true;true;true;true;true;true;true;true;true;true;true;true;true;true;true;true;true;true;true;true;true;true;true;true;true;true;true;true;true;true;true;true;true;true;true;true;true;true;true;true;true;true;true;true;true;true;true;true;true;true;true;true;true;true;true;true;true;true;true;true;true;true;true;true;true;true;true;true;true;true;true;true;true;true;true;true;true;true;true;true;true;true;true;true;true;true;true;true;true;true;true;true;true;true;true;true;true;true;true;true;true;true;true;true;true;true;true;true;true;true;true;true;true;true;true;true;true;true;true;true;true;true;true;true;true;true;true;true;true;true;true;true;true;true;true;true;true;true;true;true;true;true;true;true;true;true;true;true;true;true;true;true;true;true;true;true;true;true;true;true;true;true;true;true;true;true;true;true;true;true;true;true;true;true;true;true;true;true;true;true;true;true;true;true;true;true;true;true;true;true;true;true;true;true;true;true;true;true;true;true;true;true;true;true;true;true;true;true;true;true;true;true;true;true;true;true;true;true;true;true;true;true;true;true;true;true;true;true;true;true;true;true;true;true;true;true;true;true;true;true;true;true;true;true;true;true;true;true;true;true;true;true;true;true;true;true;true;true;true;true;true;true;true;true;true;true;true;true;true;true;true;true;true;true;true;true;true;true;true;true;true;true;true;true;true;true;true;true;true;true;true;true;true;true;true;true;true;true;true;true;true;true;true;true;true;true;true;true;true;true;true;true;true;true;true;true;true;true;true;true;true;true;true;true;true;true;true;true;true;true;true;true;true;true;true;true;true;true;true;true;true;true;true;true;true;true;true;true;true;true;true;true;true;true;true;true;true;true;true;true;true;true;true;true;true;true;true;true;true;true;true;true;true;true;true;true;true;true;true;true;true;true;true;true;true;true;true;true;true;true;true;true;true;true;true;true;true;true;true;true;true;true;true;true;true;true;true;true;true;true;true;true;true;true;true;true;true;true;true;true;true;true;true;true;true;true;true;true;true;true;true;true;true;true;true;true;true;true;true;true;true;true;true;true;true;true;true;true;true;true;true;true;true;true;true;true;true;true;true;true;true;true;true;true;true;true;true;true;true;true;true;true;true;true;true;true;true;true;true;true;true;true;true;true;true;true;true;true;true;true;true;true;true;true;true;true;true;true;true;true;true;true;true;true;true;true;true;true;true;true;true;true;true;true;true;true;true;true;true;true;true;true;true;true;true;true;true;true;true;true;true;true;true;true;true;true;true;true;true;true;true;true;true;true;true;true;true;true;true;true;true;true;true;true;true;true;true;true;true;true;true;true;true;true;true;true;true;true;true;true;true;true;true;true;true;true;true;true;true;true;true;true;true;true;true;true;true;true;true;true;true;true;true;true;true;true;true;true;true;true;true;true;true;true;true;true;true;true;true;true;true;true;true;true;true;true;true;true;true;true;true;true;true;true;true;true;true;true;true;true;true;true;true;true;true;true;true;true;true;true;true;true;true;true;true;true;true;true;true;true;true;true;true;true;true;true;true;true;true;true;true;true;true;true;true;true;true;true;true;true;true;true;true;true;true;true;true;true;true;true;true;true;true;true;true;true;true;true;true;true;true;true;true;true;true;true;true;true;true;true;true;true;true;true;true;true;true;true;true;true;true;true;true;true;true;true;true;true;true;true;true;true;true;true;true;true;true;true;true;true;true;true;true;true;true;true;true;true;true;true;true;true;true;true;true;true;true;true;true;true;true;true;true;true;true;true;true;true;true;true;true;true;true;true;true;true;true;true;true;true;true;true;true;true;true;true;true;true;true;true;true;true;true;true;true;true;true;true;true;true;true;true;true;true;true;true;true;true;true;true;true;true;true;true;true;true;true;true;true;true;true;true;true;true;true;true;true;true;true;true;true;true;true;true;true;true;true;true;true;true;true;true;true;true;true;true;true;true;true;true;true;true;true;true;true;true;true;true;true;true;true;true;true;true;true;true;true;true;true;true;true;true;true;true;true;true;true;true;true;true;true;true;true;true;true;true;true;true;true;true;true;true;true;true;true;true;true;true;true;true;true;true;true;true;true;true;true;true;true;true;true;true;true;true;true;true;true;true;true;true;true;true;true;true;true;true;true;true;true;true;true;true;true;true;true;true;true;true;true;true;true;true;true;true;true;true;true;true;true;true;true;true;true;true;true;true;true;true;true;true;true;true;true;true;true;true;true;true;true;true;true;true;true;true;true;true;true;true;true;true;true;true;true;true;true;true;true;true;true;true;true;true;true;true;true;true;true;true;true;true;true;true;true;true;true;true;true;true;true;true;true;true;true;true;true;true;true;true;true;true;true;true;true;true;true;true;true;true;true;true;true;true;true;true;true;true;true;true;true;true;true;true;true;true;true;true;true;true;true;true;true;true;true;true;true;true;true;true;true;true;true;true;true;true;true;true;true;true;true;true;true;true;true;true;true;true;true;true;true;true;true;true;true;true;true;true;true;true;true;true;true;true;true;true;true;true;true;true;true;true;true;true;true;true;true;true;true;true;true;true;true;true;true;true;true;true;true;true;true;true;true;true;true;true;true;true;true;true;true;true;true;true;true;true;true;true;true;true;true;true;true;true;true;true;true;true;true;true;true;true;true;true;true;true;true;true;true;true;true;true;true;true;true;true;true;true;true;true;true;true;true;true;true;true;true;true;true;true;true;true;true;true;true;true;true;true;true;true;true;true;true;true;true;true;true;true;true;true;true;true;true;true;true;true;true;true;true;true;true;true;true;true;true;true;true;true;true;true;true;true;true;true;true;true;true;true;true;true;true;true;true;true;true;true;true;true;true;true;true;true;true;true;true;true;true;true;true;true;true;true;true;true;true;true;true;true;true;true;true;true;true;true;true;true;true;true;true;true;true;true;true;true;true;true;true;true;true;true;true;true;true;true;true;true;true;true;true;true;true;true;true;true;true;true;true;true;true;true;true;true;true;true;true;true;true;true;true;true;true;true;true;true;true;true;true;true;true;true;true;true;true;true;true;true;true;true;true;true;true;true;true;true;true;true;true;true;true;true;true;true;true;true;true;true;true;true;true;true;true;true;true;true;true;true;true;true;true;true;true;true;true;true;true;true;true;true;true;true;true;true;true;true;true;true;true;true;true;true;true;true;true;true;true;true;true;true;true;true;true;true;true;true;true;true;true;true;true;true;true;true;true;true;true;true;true;true;true;true;true;true;true;true;true;true;true;true;true;true;true;true;true;true;true;true;true;true;true;true;true;true;true;true;true;true;true;true;true;true;true;true;true;true;true;true;true;true;true;true;true;true;true;true;true;true;true;true;true;true;true;true;true;true;true;true;true;true;true;true;true;true;true;true;true;true;true;true;true;true;true;true;true;true;true;true;true;true;true;true;true;true;true;true;true;true;true;true;true;true;true;true;true;true;true;true;true;true;true;true;true;true;true;true;true;true;true;true;true;true;true;true;true;true;true;true;true;true;true;true;true;true;true;true;true;true;true;true;true;true;true;true;true;true;true;true;true;true;true;true;true;true;true;true;true;true;true;true;true;true;true;true;true;true;true;true;true;true;true;true;true;true;true;true;true;true;true;true;true;true;true;true;true;true;true;true;true;true;true;true;true;true;true;true;true;true;true;true;true;true;true;true;true;true;true;true;true;true;true;true;true;true;true;true;true;true;true;true;true;true;true;true;true;true;true;true;true;true;true;true;true;true;true;true;true;true;true;true;true;true;true;true;true;true;true;true;true;true;true;true;true;true;true;true;true;true;true;true;true;true;true;true;true;true;true;true;true;true;true;true;true;true;true;true;true;true;true;true;true;true;true;true;true;true;true;true;true;true;true;true;true;true;true;true;true;true;true;true;true;true;true;true;true;true;true;true;true;true;true;true;true;true;true;true;true;true;true;true;true;true;true;true;true;true;true;true;true;true;true;true;true;true;true;true;true;true;true;true;true;true;true;true;true;true;true;true;true;true;true;true;true;true;true;true;true;true;true;true;true;true;true;true;true;true;true;true;true;true;true;true;true;true;true;true;true;true;true;true;true;true;true;true;true;true;true;true;true;true;true;true;true;true;true;true;true;true;true;true;true;true;true;true;true;true;true;true;true;true;true;true;true;true;true;true;true;true;true;true;true;true;true;true;true;true;true;true;true;true;true;true;true;true;true;true;true;true;true;true;true;true;true;true;true;true;true;true;true;true;true;true;true;true;true;true;true;true;true;true;true;true;true;true;true;true;true;true;true;true;true;true;true;true;true;true;true;true;true;true;true;true;true;true;true;true;true;true;true;true;true;true;true;true;true;true;true;true;true;true;true;true;true;true;true;true;true;true;true;true;true;true;true;true;true;true;true;true;true;true;true;true;true;true;true;true;true;true;true;true;true;true;true;true;true;true;true;true;true;true;true;true;true;true;true;true;true;true;true;true;true;true;true;true;true;true;true;true;true;true;true;true;true;true;true;true;true;true;true;true;true;true;true;true;true;true;true;true;true;true;true;true;true;true;true;true;true;true;true;true;true;true;true;true;true;true;true;true;true;true;true;true;true;true;true;true;true;true;true;true;true;true;true;true;true;true;true;true;true;true;true;true;true;true;true;true;true;true;true;true;true;true;true;true;true;true;true;true;true;true;true;true;true;true;true;true;true;true;true;true;true;true;true;true;true;true;true;true;true;true;true;true;true;true;true;true;true;true;true;true;true;true;true;true;true;true;true;true;true;true;true;true;true;true;true;true;true;true;true;true;true;true;true;true;true;true;true;true;true;true;true;true;true;true;true;true;true;true;true;true;true;true;true;true;true;true;true;true;true;true;true;true;true;true;true;true;true;true;true;true;true;true;true;true;true;true;true;true;true;true;true;true;true;true;true;true;true;true;true;true;true;true;true;true;true;true;true;true;true;true;true;true;true;true;true;true;true;true;true;true;true;true;true;true;true;true;true;true;true;true;true;true;true;true;true;true;true;true;true;true;true;true;true;true;true;true;true;true;true;true;true;true;true;true;true;true;true;true;true;true;true;true;true;true;true;true;true;true;true;true;true;true;true;true;true;true;true;true;true;true;true;true;true;true;true;true;true;true;true;true;true;true;true;true;true;true;true;true;true;true;true;true;true;true;true;true;true;true;true;true;true;true;true;true;true;true;true;true;true;true;true;true;true;true;true;true;true;true;true;true;true;true;true;true;true;true;true;true;true;true;true;true;true;true;true;true;true;true;true;true;true;true;true;true;true;true;true;true;true;true;true;true;true;true;true;true;true;true;true;true;true;true;true;true;true;true;true;true;true;true;true;true;true;true;true;true;true;true;true;true;true;true;true;true;true;true;true;true;true;true;true;true;true;true;true;true;true;true;true;true;true;true;true;true;true;true;true;true;true;true;true;true;true;true;true;true;true;true;true;true;true;true;true;true;true;true;true;true;true;true;true;true;true;true;true;true;true;true;true;true;true;true;true;true;true;true;true;true;true;true;true;true;true;true;true;true;true;true;true;true;true;true;true;true;true;true;true;true;true;true;true;true;true;true;true;true;true;true;true;true;true;true;true;true;true;true;true;true;true;true;true;true;true;true;true;true;true;true;true;true;true;true;true;true;true;true;true;true;true;true;true;true;true;true;true;true;true;true;true;true;true;true;true;true;true;true;true;true;true;true;true;true;true;true;true;true;true;true;true;true;true;true;true;true;true;true;true;true;true;true;true;true;true;true;true;true;true;true;true;true;true;true;true;true;true;true;true;true;true;true;true;true;true;true;true;true;true;true;true;true;true;true;true;true;true;true;true;true;true;true;true;true;true;true;true;true;true;true;true;true;true;true;true;true;true;true;true;true;true;true;true;true;true;true;true;true;true;true;true;true;true;true;true;true;true;true;true;true;true;true;true;true;true;true;true;true;true;true;true;true;true;true;true;true;true;true;true;true;true;true;true;true;true;true;true;true;true;true;true;true;true;true;true;true;true;true;true;true;true;true;true;true;true;true;true;true;true;true;true;true;true;true;true;true;true;true;true;true;true;true;true;true;true;true;true;true;true;true;true;true;true;true;true;true;true;true;true;true;true;true;true;true;true;true;true;true;true;true;true;true;true;true;true;true;true;true;true;true;true;true;true;true;true;true;true;true;true;true;true;true;true;true;true;true;true;true;true;true;true;true;true;true;true;true;true;true;true;true;true;true;true;true;true;true;true;true;true;true;true;true;true;true;true;true;true;true;true;true;true;true;true;true;true;true;true;true;true;true;true;true;true;true;true;true;true;true;true;true;true;true;true;true;true;true;true;true;true;true;true;true;true;true;true;true;true;true;true;true;true;true;true;true;true;true;true;true;true;true;true;true;true;true;true;true;true;true;true;true;true;true;true;true;true;true;true;true;true;true;true;true;true;true;true;true;true;true;true;true;true;true;true;true;true;true;true;true;true;true;true;true;true;true;true;true;true;true;true;true;true;true;true;true;true;true;true;true;true;true;true;true;true;true;true;true;true;true;true;true;true;true;true;true;true;true;true;true;true;true;true;true;true;true;true;true;true;true;true;true;true;true;true;true;true;true;true;true;true;true;true;true;true;true;true;true;true;true;true;true;true;true;true;true;true;true;true;true;true;true;true;true;true;true;true;true;true;true;true;true;true;true;true;true;true;true;true;true;true;true;true;true;true;true;true;true;true;true;true;true;true;true;true;true;true;true;true;true;true;true;true;true;true;true;true;true;true;true;true;true;true;true;true;true;true;true;true;true;true;true;true;true;true;true;true;true;true;true;true;true;true;true;true;true;true;true;true;true;true;true;true;true;true;true;true;true;true;true;true;true;true;true;true;true;true;true;true;true;true;true;true;true;true;true;true;true;true;true;true;true;true;true;true;true;true;true;true;true;true;true;true;true;true;true;true;true;true;true;true;true;true;true;true;true;true;true;true;true;true;true;true;true;true;true;true;true;true;true;true;true;true;true;true;true;true;true;true;true;true;true;true;true;true;true;true;true;true;true;true;true;true;true;true;true;true;true;true;true;true;true;true;true;true;true;true;true;true;true;true;true;true;true;true;true;true;true;true;true;true;true;true;true;true;true;true;true;true;true;true;true;true;true;true;true;true;true;true;true;true;true;true;true;true;true;true;true;true;true;true;true;true;true;true;true;true;true;true;true;true;true;true;true;true;true;true;true;true;true;true;true;true;true;true;true;true;true;true;true;true;true;true;true;true;true;true;true;true;true;true;true;true;true;true;true;true;true;true;true;true;true;true;true;true;true;true;true;true;true;true;true;true;true;true;true;true;true;true;true;true;true;true;true;true;true;true;true;true;true;true;true;true;true;true;true;true;true;true;true;true;true;true;true;true;true;true;true;true;true;true;true;true;true;true;true;true;true;true;true;true;true;true;true;true;true;true;true;true;true;true;true;true;true;true;true;true;true;true;true;true;true;true;true;true;true;true;true;true;true;true;true;true;true;true;true;true;true;true;true;true;true;true;true;true;true;true;true;true;true;true;true;true;true;true;true;true;true;true;true;true;true;true;true;true;true;true;true;true;true;true;true;true;true;true;true;true;true;true;true;true;true;true;true;true;true;true;true;true;true;true;true;true;true;true;true;true;true;true;true;true;true;true;true;true;true;true;true;true;true;true;true;true;true;true;true;true;true;true;true;true;true;true;true;true;true;true;true;true;true;true;true;true;true;true;true;true;true;true;true;true;true;true;true;true;true;true;true;true;true;true;true;true;true;true;true;true;true;true;true;true;true;true;true;true;true;true;true;true;true;true;true;true;true;true;true;true;true;true;true;true;true;true;true;true;true;true;true;true;true;true;true;true;true;true;true;true;true;true;true;true;true;true;true;true;true;true;true;true;true;true;true;true;true;true;true;true;true;true;true;true;true;true;true;true;true;true;true;true;true;true;true;true;true;true;true;true;true;true;true;true;true;true;true;true;true;true;true;true;true;true;true;true;true;true;true;true;true;true;true;true;true;true;true;true;true;true;true;true;true;true;true;true;true;true;true;true;true;true;true;true;true;true;true;true;true;true;true;true;true;true;true;true;true;true;true;true;true;true;true;true;true;true;true;true;true;true;true;true;true;true;true;true;true;true;true;true;true;true;true;true;true;true;true;true;true;true;true;true;true;true;true;true;true;true;true;true;true;true;true;true;true;true;true;true;true;true;true;true;true;true;true;true;true;true;true;true;true;true;true;true;true;true;true;true;true;true;true;true;true;true;true;true;true;true;true;true;true;true;true;true;true;true;true;true;true;true;true;true;true;true;true;true;true;true;true;true;true;true;true;true;true;true;true;true;true;true;true;true;true;true;true;true;true;true;true;true;true;true;true;true;true;true;true;true;true;true;true;true;true;true;true;true;true;true;true;true;true;true;true;true;true;true;true;true;true;true;true;true;true;true;true;true;true;true;true;true;true;true;true;true;true;true;true;true;true;true;true;true;true;true;true;true;true;true;true;true;true;true;true;true;true;true;true;true;true;true;true;true;true;true;true;true;true;true;true;true;true;true;true;true;true;true;true;true;true;true;true;true;true;true;true;true;true;true;true;true;true;true;true;true;true;true;true;true;true;true;true;true;true;true;true;true;true;true;true;true;true;true;true;true;true;true;true;true;true;true;true;true;true;true;true;true;true;true;true;true;true;true;true;true;true;true;true;true;true;true;true;true;true;true;true;true;true;true;true;true;true;true;true;true;true;true;true;true;true;true;true;true;true;true;true;true;true;true;true;true;true;true;true;true;true;true;true;true;true;true;true;true;true;true;true;true;true;true;true;true;true;true;true;true;true;true;true;true;true;true;true;true;true;true;true;true;true;true;true;true;true;true;true;true;true;true;true;true;true;true;true;true;true;true;true;true;true;true;true;true;true;true;true;true;true;true;true;true;true;true;true;true;true;true;true;true;true;true;true;true;true;true;true;true;true;true;true;true;true;true;true;true;true;true;true;true;true;true;true;true;true;true;true;true;true;true;true;true;true;true;true;true;true;true;true;true;true;true;true;true;true;true;true;true;true;true;true;true;true;true;true;true;true;true;true;true;true;true;true;true;true;true;true;true;true;true;true;true;true;true;true;true;true;true;true;true;true;true;true;true;true;true;true;true;true;true;true;true;true;true;true;true;true;true;true;true;true;true;true;true;true;true;true;true;true;true;true;true;true;true;true;true;true;true;true;true;true;true;true;true;true;true;true;true;true;true;true;true;true;true;true;true;true;true;true;true;true;true;true;true;true;true;true;true;true;true;true;true;true;true;true;true;true;true;true;true;true;true;true;true;true;true;true;true;true;true;true;true;true;true;true;true;true;true;true;true;true;true;true;true;true;true;true;true;true;true;true;true;true;true;true;true;true;true;true;true;true;true;true;true;true;true;true;true;true;true;true;true;true;true;true;true;true;true;true;true;true;true;true;true;true;true;true;true;true;true;true;true;true;true;true;true;true;true;true;true;true;true;true;true;true;true;true;true;true;true;true;true;true;true;true;true;true;true;true;true;true;true;true;true;true;true;true;true;true;true;true;true;true;true;true;true;true;true;true;true;true;true;true;true;true;true;true;true;true;true;true;true;true;true;true;true;true;true;true;true;true;true;true;true;true;true;true;true;true;true;true;true;true;true;true;true;true;true;true;true;true;true;true;true;true;true;true;true;true;true;true;true;true;true;true;true;true;true;true;true;true;true;true;true;true;true;true;true;true;true;true;true;true;true;true;true;true;true;true;true;true;true;true;true;true;true;true;true;true;true;true;true;true;true;true;true;true;true;true;true;true;true;true;true;true;true;true;true;true;true;true;true;true;true;true;true;true;true;true;true;true;true;true;true;true;true;true;true;true;true;true;true;true;true;true;true;true;true;true;true;true;true;true;true;true;true;true;true;true;true;true;true;true;true;true;true;true;true;true;true;true;true;true;true;true;true;true;true;true;true;true;true;true;true;true;true;true;true;true;true;true;true;true;true;true;true;true;true;true;true;true;true;true;true;true;true;true;true;true;true;true;true;true;true;true;true;true;true;true;true;true;true;true;true;true;true;true;true;true;true;true;true;true;true;true;true;true;true;true;true;true;true;true;true;true;true;true;true;true;true;true;true;true;true;true;true;true;true;true;true;true;true;true;true;true;true;true;true;true;true;true;true;true;true;true;true;true;true;true;true;true;true;true;true;true;true;true;true;true;true;true;true;true;true;true;true;true;true;true;true;true;true;true;true;true;true;true;true;true;true;true;true;true;true;true;true;true;true;true;true;true;true;true;true;true;true;true;true;true;true;true;true;true;true;true;true;true;true;true;true;true;true;true;true;true;true;true;true;true;true;true;true;true;true;true;true;true;true;true;true;true;true;true;true;true;true;true;true;true;true;true;true;true;true;true;true;true;true;true;true;true;true;true;true;true;true;true;true;true;true;true;true;true;true;true;true;true;true;true;true;true;true;true;true;true;true;true;true;true;true;true;true;true;true;true;true;true;true;true;true;true;true;true;true;true;true;true;true;true;true;true;true;true;true;true;true;true;true;true;true;true;true;true;true;true;true;true;true;true;true;true;true;true;true;true;true;true;true;true;true;true;true;true;true;true;true;true;true;true;true;true;true;true;true;true;true;true;true;true;true;true;true;true;true;true;true;true;true;true;true;true;true;true;true;true;true;true;true;true;true;true;true;true;true;true;true;true;true;true;true;true;true;true;true;true;true;true;true;true;true;true;true;true;true;true;true;true;true;true;true;true;true;true;true;true;true;true;true;true;true;true;true;true;true;true;true;true;true;true;true;true;true;true;true;true;true;true;true;true;true;true;true;true;true;true;true;true;true;true;true;true;true;true;true;true;true;true;true;true;true;true;true;true;true;true;true;true;true;true;true;true;true;true;true;true;true;true;true;true;true;true;true;true;true;true;true;true;true;true;true;true;true;true;true;true;true;true;true;true;true;true;true;true;true;true;true;true;true;true;true;true;true;true;true;true;true;true;true;true;true;true;true;true;true;true;true;true;true;true;true;true;true;true;true;true;true;true;true;true;true;true;true;true;true;true;true;true;true;true;true;true;true;true;true;true;true;true;true;true;true;true;true;true;true;true;true;true;true;true;true;true;true;true;true;true;true;true;true;true;true;true;true;true;true;true;true;true;true;true;true;true;true;true;true;true;true;true;true;true;true;true;true;true;true;true;true;true;true;true;true;true;true;true;true;true;true;true;true;true;true;true;true;true;true;true;true;true;true;true;true;true;true;true;true;true;true;true;true;true;true;true;true;true;true;true;true;true;true;true;true;true;true;true;true;true;true;true;true;true;true;true;true;true;true;true;true;true;true;true;true;true;true;true;true;true;true;true;true;true;true;true;true;true;true;true;true;true;true;true;true;true;true;true;true;true;true;true;true;true;true;true;true;true;true;true;true;true;true;true;true;true;true;true;true;true;true;true;true;true;true;true;true;true;true;true;true;true;true;true;true;true;true;true;true;true;true;true;true;true;true;true;true;true;true;true;true;true;true;true;true;true;true;true;true;true;true;true;true;true;true;true;true;true;true;true;true;true;true;true;true;true;true;true;true;true;true;true;true;true;true;true;true;true;true;true;true;true;true;true;true;true;true;true;true;true;true;true;true;true;true;true;true;true;true;true;true;true;true;true;true;true;true;true;true;true;true;true;true;true;true;true;true;true;true;true;true;true;true;true;true;true;true;true;true;true;true;true;true;true;true;true;true;true;true;true;true;true;true;true;true;true;true;true;true;true;true;true;true;true;true;true;true;true;true;true;true;true;true;true;true;true;true;true;true;true;true;true;true;true;true;true;true;true;true;true;true;true;true;true;true;true;true;true;true;true;true;true;true;true;true;true;true;true;true;true;true;true;true;true;true;true;true;true;true;true;true;true;true;true;true;true;true;true;true;true;true;true;true;true;true;true;true;true;true;true;true;true;true;true;true;true;true;true;true;true;true;true;true;true;true;true;true;true;true;true;true;true;true;true;true;true;true;true;true;true;true;true;true;true;true;true;true;true;true;true;true;true;true;true;true;true;true;true;true;true;true;true;true;true;true;true;true;true;true;true;true;true;true;true;true;true;true;true;true;true;true;true;true;true;true;true;true;true;true;true;true;true;true;true;true;true;true;true;true;true;true;true;true;true;true;true;true;true;true;true;true;true;true;true;true;true;true;true;true;true;true;true;true;true;true;true;true;true;true;true;true;true;true;true;true;true;true;true;true;true;true;true;true;true;true;true;true;true;true;true;true;true;true;true;true;true;true;true;true;true;true;true;true;true;true;true;true;true;true;true;true;true;true;true;true;true;true;true;true;true;true;true;true;true;true;true;true;true;true;true;true;true;true;true;true;true;true;true;true;true;true;true;true;true;true;true;true;true;true;true;true;true;true;true;true;true;true;true;true;true;true;true;true;true;true;true;true;true;true;true;true;true;true;true;true;true;true;true;true;true;true;true;true;true;true;true;true;true;true;true;true;true;true;true;true;true;true;true;true;true;true;true;true;true;true;true;true;true;true;true;true;true;true;true;true;true;true;true;true;true;true;true;true;true;true;true;true;true;true;true;true;true;true;true;true;true;true;true;true;true;true;true;true;true;true;true;true;true;true;true;true;true;true;true;true;true;true;true;true;true;true;true;true;true;true;true;true;true;true;true;true;true;true;true;true;true;true;true;true;true;true;true;true;true;true;true;true;true;true;true;true;true;true;true;true;true;true;true;true;true;true;true;true;true;true;true;true;true;true;true;true;true;true;true;true;true;true;true;true;true;true;true;true;true;true;true;true;true;true;true;true;true;true;true;true;true;true;true;true;true;true;true;true;true;true;true;true;true;true;true;true;true;true;true;true;true;true;true;true;true;true;true;true;true;true;true;true;true;true;true;true;true;true;true;true;true;true;true;true;true;true;true;true;true;true;true;true;true;true;true;true;true;true;true;true;true;true;true;true;true;true;true;true;true;true;true;true;true;true;true;true;true;true;true;true;true;true;true;true;true;true;true;true;true;true;true;true;true;true;true;true;true;true;true;true;true;true;true;true;true;true;true;true;true;true;true;true;true;true;true;true;true;true;true;true;true;true;true;true;true;true;true;true;true;true;true;true;true;true;true;true;true;true;true;true;true;true;true;true;true;true;true;true;true;true;true;true;true;true;true;true;true;true;true;true;true;true;true;true;true;true;true;true;true;true;true;true;true;true;true;true;true;true;true;true;true;true;true;true;true;true;true;true;true;true;true;true;true;true;true;true;true;true;true;true;true;true;true;true;true;true;true;true;true;true;true;true;true;true;true;true;true;true;true;true;true;true;true;true;true;true;true;true;true;true;true;true;true;true;true;true;true;true;true;true;true;true;true;true;true;true;true;true;true;true;true;true;true;true;true;true;true;true;true;true;true;true;true;true;true;true;true;true;true;true;true;true;true;true;true;true;true;true;true;true;true;true;true;true;true;true;true;true;true;true;true;true;true;true;true;true;true;true;true;true;true;true;true;true;true;true;true;true;true;true;true;true;true;true;true;true;true;true;true;true;true;true;true;true;true;true;true;true;true;true;true;true;true;true;true;true;true;true;true;true;true;true;true;true;true;true;true;true;true;true;true;true;true;true;true;true;true;true;true;true;true;true;true;true;true;true;true;true;true;true;true;true;true;true;true;true;true;true;true;true;true;true;true;true;true;true;true;true;true;true;true;true;true;true;true;true;true;true;true;true;true;true;true;true;true;true;true;true;true;true;true;true;true;true;true;true;true;true;true;true;true;true;true;true;true;true;true;true;true;true;true;true;true;true;true;true;true;true;true;true;true;true;true;true;true;true;true;true;true;true;true;true;true;true;true;true;true;true;true;true;true;true;true;true;true;true;true;true;true;true;true;true;true;true;true;true;true;true;true;true;true;true;true;true;true;true;true;true;true;true;true;true;true;true;true;true;true;true;true;true;true;true;true;true;true;true;true;true;true;true;true;true;true;true;true;true;true;true;true;true;true;true;true;true;true;true;true;true;true;true;true;true;true;true;true;true;true;true;true;true;true;true;true;true;true;true;true;true;true;true;true;true;true;true;true;true;true;true;true;true;true;true;true;true;true;true;true;true;true;true;true;true;true;true;true;true;true;true;true;true;true;true;true;true;true;true;true;true;true;true;true;true;true;true;true;true;true;true;true;true;true;true;true;true;true;true;true;true;true;true;true;true;true;true;true;true;true;true;true;true;true;true;true;true;true;true;true;true;true;true;true;true;true;true;true;true;true;true;true;true;true;true;true;true;true;true;true;true;true;true;true;true;true;true;true;true;true;true;true;true;true;true;true;true;true;true;true;true;true;true;true;true;true;true;true;true;true;true;true;true;true;true;true;true;true;true;true;true;true;true;true;true;true;true;true;true;true;true;true;true;true;true;true;true;true;true;true;true;true;true;true;true;true;true;true;true;true;true;true;true;true;true;true;true;true;true;true;true;true;true;true;true;true;true;true;true;true;true;true;true;true;true;true;true;true;true;true;true;true;true;true;true;true;true;true;true;true;true;true;true;true;true;true;true;true;true;true;true;true;true;true;true;true;true;true;true;true;true;true;true;true;true;true;true;true;true;true;true;true;true;true;true;true;true;true;true;true;true;true;true;true;true;true;true;true;true;true;true;true;true;true;true;true;true;true;true;true;true;true;true;true;true;true;true;true;true;true;true;true;true;true;true;true;true;true;true;true;true;true;true;true;true;true;true;true;true;true;true;true;true;true;true;true;true;true;true;true;true;true;true;true;true;true;true;true;true;true;true;true;true;true;true;true;true;true;true;true;true;true;true;true;true;true;true;true;true;true;true;true;true;true;true;true;true;true;true;true;true;true;true;true;true;true;true;true;true;true;true;true;true;true;true;true;true;true;true;true;true;true;true;true;true;true;true;true;true;true;true;true;true;true;true;true;true;true;true;true;true;true;true;true;true;true;true;true;true;true;true;true;true;true;true;true;true;true;true;true;true;true;true;true;true;true;true;true;true;true;true;true;true;true;true;true;true;true;true;true;true;true;true;true;true;true;true;true;true;true;true;true;true;true;true;true;true;true;true;true;true;true;true;true;true;true;true;true;true;true;true;true;true;true;true;true;true;true;true;true;true;true;true;true;true;true;true;true;true;true;true;true;true;true;true;true;true;true;true;true;true;true;true;true;true;true;true;true;true;true;true;true;true;true;true;true;true;true;true;true;true;true;true;true;true;true;true;true;true;true;true;true;true;true;true;true;true;true;true;true;true;true;true;true;true;true;true;true;true;true;true;true;true;true;true;true;true;true;true;true;true;true;true;true;true;true;true;true;true;true;true;true;true;true;true;true;true;true;true;true;true;true;true;true;true;true;true;true;true;true;true;true;true;true;true;true;true;true;true;true;true;true;true;true;true;true;true;true;true;true;true;true;true;true;true;true;true;true;true;true;true;true;true;true;true;true;true;true;true;true;true;true;true;true;true;true;true;true;true;true;true;true;true;true;true;true;true;true;true;true;true;true;true;true;true;true;true;true;true;true;true;true;true;true;true;true;true;true;true;true;true;true;true;true;true;true;true;true;true;true;true;true;true;true;true;true;true;true;true;true;true;true;true;true;true;true;true;true;true;true;true;true;true;true;true;true;true;true;true;true;true;true;true;true;true;true;true;true;true;true;true;true;true;true;true;true;true;true;true;true;true;true;true;true;true;true;true;true;true;true;true;true;true;true;true;true;true;true;true;true;true;true;true;true;true;true;true;true;true;true;true;true;true;true;true;true;true;true;true;true;true;true;true;true;true;true;true;true;true;true;true;true;true;true;true;true;true;true;true;true;true;true;true;true;true;true;true;true;true;true;true;true;true;true;true;true;true;true;true;true;true;true;true;true;true;true;true;true;true;true;true;true;true;true;true;true;true;true;true;true;true;true;true;true;true;true;true;true;true;true;true;true;true;true;true;true;true;true;true;true;true;true;true;true;true;true;true;true;true;true;true;true;true;true;true;true;true;true;true;true;true;true;true;true;true;true;true;true;true;true;true;true;true;true;true;true;true;true;true;true;true;true;true;true;true;true;true;true;true;true;true;true;true;true;true;true;true;true;true;true;true;true;true;true;true;true;true;true;true;true;true;true;true;true;true;true;true;true;true;true;true;true;true;true;true;true;true;true;true;true;true;true;true;true;true;true;true;true;true;true;true;true;true;true;true;true;true;true;true;true;true;true;true;true;true;true;true;true;true;true;true;true;true;true;true;true;true;true;true;true;true;true;true;true;true;true;true;true;true;true;true;true;true;true;true;true;true;true;true;true;true;true;true;true;true;true;true;true;true;true;true;true;true;true;true;true;true;true;true;true;true;true;true;true;true;true;true;true;true;true;true;true;true;true;true;true;true;true;true;true;true;true;true;true;true;true;true;true;true;true;true;true;true;true;true;true;true;true;true;true;true;true;true;true;true;true;true;true;true;true;true;true;true;true;true;true;true;true;true;true;true;true;true;true;true;true;true;true;true;true;true;true;true;true;true;true;true;true;true;true;true;true;true;true;true;true;true;true;true;true;true;true;true;true;true;true;true;true;true;true;true;true;true;true;true;true;true;true;true;true;true;true;true;true;true;true;true;true;true;true;true;true;true;true;true;true;true;true;true;true;true;true;true;true;true;true;true;true;true;true;true;true;true;true;true;true;true;true;true;true;true;true;true;true;true;true;true;true;true;true;true;true;true;true;true;true;true;true;true;true;true;true;true;true;true;true;true;true;true;true;true;true;true;true;true;true;true;true;true;true;true;true;true;true;true;true;true;true;true;true;true;true;true;true;true;true;true;true;true;true;true;true;true;true;true;true;true;true;true;true;true;true;true;true;true;true;true;true;true;true;true;true;true;true;true;true;true;true;true;true;true;true;true;true;true;true;true;true;true;true;true;true;true;true;true;true;true;true;true;true;true;true;true;true;true;true;true;true;true;true;true;true;true;true;true;true;true;true;true;true;true;true;true;true;true;true;true;true;true;true;true;true;true;true;true;true;true;true;true;true;true;true;true;true;true;true;true;true;true;true;true;true;true;true;true;true;true;true;true;true;true;true;true;true;true;true;true;true;true;true;true;true;true;true;true;true;true;true;true;true;true;true;true;true;true;true;true;true;true;true;true;true;true;true;true;true;true;true;true;true;true;true;true;true;true;true;true;true;true;true;true;true;true;true;true;true;true;true;true;true;true;true;true;true;true;true;true;true;true;true;true;true;true;true;true;true;true;true;true;true;true;true;true;true;true;true;true;true;true;true;true;true;true;true;true;true;true;true;true;true;true;true;true;true;true;true;true;true;true;true;true;true;true;true;true;true;true;true;true;true;true;true;true;true;true;true;true;true;true;true;true;true;true;true;true;true;true;true;true;true;true;true;true;true;true;true;true;true;true;true;true;true;true;true;true;true;true;true;true;true;true;true;true;true;true;true;true;true;true;true;true;true;true;true;true;true;true;true;true;true;true;true;true;true;true;true;true;true;true;true;true;true;true;true;true;true;true;true;true;true;true;true;true;true;true;true;true;true;true;true;true;true;true;true;true;true;true;true;true;true;true;true;true;true;true;true;true;true;true;true;true;true;true;true;true;true;true;true;true;true;true;true;true;true;true;true;true;true;true;true;true;true;true;true;true;true;true;true;true;true;true;true;true;true;true;true;true;true;true;true;true;true;true;true;true;true;true;true;true;true;true;true;true;true;true;true;true;true;true;true;true;true;true;true;true;true;true;true;true;true;true;true;true;true;true;true;true;true;true;true;true;true;true;true;true;true;true;true;true;true;true;true;true;true;true;true;true;true;true;true;true;true;true;true;true;true;true;true;true;true;true;true;true;true;true;true;true;true;true;true;true;true;true;true;true;true;true;true;true;true;true;true;true;true;true;true;true;true;true;true;true;true;true;true;true;true;true;true;true;true;true;true;true;true;true;true;true;true;true;true;true;true;true;true;true;true;true;true;true;true;true;true;true;true;true;true;true;true;true;true;true;true;true;true;true;true;true;true;true;true;true;true;true;true;true;true;true;true;true;true;true;true;true;true;true;true;true;true;true;true;true;true;true;true;true;true;true;true;true;true;true;true;true;true;true;true;true;true;true;true;true;true;true;true;true;true;true;true;true;true;true;true;true;true;true;true;true;true;true;true;true;true;true;true;true;true;true;true;true;true;true;true;true;true;true;true;true;true;true;true;true;true;true;true;true;true;true;true;true;true;true;true;true;true;true;true;true;true;true;true;true;true;true;true;true;true;true;true;true;true;true;true;true;true;true;true;true;true;true;true;true;true;true;true;true;true;true;true;true;true;true;true;true;true;true;true;true;true;true;true;true;true;true;true;true;true;true;true;true;true;true;true;true;true;true;true;true;true;true;true;true;true;true;true;true;true;true;true;true;true;true;true;true;true;true;true;true;true;true;true;true;true;true;true;true;true;true;true;true;true;true;true;true;true;true;true;true;true;true;true;true;true;true;true;true;true;true;true;true;true;true;true;true;true;true;true;true;true;true;true;true;true;true;true;true;true;true;true;true;true;true;true;true;true;true;true;true;true;true;true;true;true;true;true;true;true;true;true;true;true;true;true;true;true;true;true;true;true;true;true;true;true;true;true;true;true;true;true;true;true;true;true;true;true;true;true;true;true;true;true;true;true;true;true;true;true;true;true;true;true;true;true;true;true;true;true;true;true;true;true;true;true;true;true;true;true;true;true;true;true;true;true;true;true;true;true;true;true;true;true;true;true;true;true;true;true;true;true;true;true;true;true;true;true;true;true;true;true;true;true;true;true;true;true;true;true;true;true;true;true;true;true;true;true;true;true;true;true;true;true;true;true;true;true;true;true;true;true;true;true;true;true;true;true;true;true;true;true;true;true;true;true;true;true;true;true;true;true;true;true;true;true;true;true;true;true;true;true;true;true;true;true;true;true;true;true;true;true;true;true;true;true;true;true;true;true;true;true;true;true;true;true;true;true;true;true;true;true;true;true;true;true;true;true;true;true;true;true;true;true;true;true;true;true;true;true;true;true;true;true;true;true;true;true;true;true;true;true;true;true;true;true;true;true;true;true;true;true;true;true;true;true;true;true;true;true;true;true;true;true;true;true;true;true;true;true;true;true;true;true;true;true;true;true;true;true;true;true;true;true;true;true;true;true;true;true;true;true;true;true;true;true;true;true;true;true;true;true;true;true;true;true;true;true;true;true;true;true;true;true;true;true;true;true;true;true;true;true;true;true;true;true;true;true;true;true;true;true;true;true;true;true;true;true;true;true;true;true;true;true;true;true;true;true;true;true;true;true;true;true;true;true;true;true;true;true;true;true;true;true;true;true;true;true;true;true;true;true;true;true;true;true;true;true;true;true;true;true;true;true;true;true;true;true;true;true;true;true;true;true;true;true;true;true;true;true;true;true;true;true;true;true;true;true;true;true;true;true;true;true;true;true;true;true;true;true;true;true;true;true;true;true;true;true;true;true;true;true;true;true;true;true;true;true;true;true;true;true;true;true;true;true;true;true;true;true;true;true;true;true;true;true;true;true;true;true;true;true;true;true;true;true;true;true;true;true;true;true;true;true;true;true;true;true;true;true;true;true;true;true;true;true;true;true;true;true;true;true;true;true;true;true;true;true;true;true;true;true;true;true;true;true;true;true;true;true;true;true;true;true;true;true;true;true;true;true;true;true;true;true;true;true;true;true;true;true;true;true;true;true;true;true;true;true;true;true;true;true;true;true;true;true;true;true;true;true;true;true;true;true;true;true;true;true;true;true;true;true;true;true;true;true;true;true;true;true;true;true;true;true;true;true;true;true;true;true;true;true;true;true;true;true;true;true;true;true;true;true;true;true;true;true;true;true;true;true;true;true;true;true;true;true;true;true;true;true;true;true;true;true;true;true;true;true;true;true;true;true;true;true;true;true;true;true;true;true;true;true;true;true;true;true;true;true;true;true;true;true;true;true;true;true;true;true;true;true;true;true;true;true;true;true;true;true;true;true;true;true;true;true;true;true;true;true;true;true;true;true;true;true;true;true;true;true;true;true;true;true;true;true;true;true;true;true;true;true;true;true;true;true;true;true;true;true;true;true;true;true;true;true;true;true;true;true;true;true;true;true;true;true;true;true;true;true;true;true;true;true;true;true;true;true;true;true;true;true;true;true;true;true;true;true;true;true;true;true;true;true;true;true;true;true;true;true;true;true;true;true;true;true;true;true;true;true;true;true;true;true;true;true;true;true;true;true;true;true;true;true;true;true;true;true;true;true;true;true;true;true;true;true;true;true;true;true;true;true;true;true;true;true;true;true;true;true;true;true;true;true;true;true;true;true;true;true;true;true;true;true;true;true;true;true;true;true;true;true;true;true;true;true;true;true;true;true;true;true;true;true;true;true;true;true;true;true;true;true;true;true;true;true;true;true;true;true;true;true;true;true;true;true;true;true;true;true;true;true;true;true;true;true;true;true;true;true;true;true;true;true;true;true;true;true;true;true;true;true;true;true;true;true;true;true;true;true;true;true;true;true;true;true;true;true;true;true;true;true;true;true;true;true;true;true;true;true;true;true;true;true;true;true;true;true;true;true;true;true;true;true;true;true;true;true;true;true;true;true;true;true;true;true;true;true;true;true;true;true;true;true;true;true;true;true;true;true;true;true;true;true;true;true;true;true;true;true;true;true;true;true;true;true;true;true;true;true;true;true;true;true;true;true;true;true;true;true;true;true;true;true;true;true;true;true;true;true;true;true;true;true;true;true;true;true;true;true;true;true;true;true;true;true;true;true;true;true;true;true;true;true;true;true;true;true;true;true;true;true;true;true;true;true;true;true;true;true;true;true;true;true;true;true;true;true;true;true;true;true;true;true;true;true;true;true;true;true;true;true;true;true;true;true;true;true;true;true;true;true;true;true;true;true;true;true;true;true;true;true;true;true;true;true;true;true;true;true;true;true;true;true;true;true;true;true;true;true;true;true;true;true;true;true;true;true;true;true;true;true;true;true;true;true;true;true;true;true;true;true;true;true;true;true;true;true;true;true;true;true;true;true;true;true;true;true;true;true;true;true;true;true;true;true;true;true;true;true;true;true;true;true;true;true;true;true;true;true;true;true;true;true;true;true;true;true;true;true;true;true;true;true;true;true;true;true;true;true;true;true;true;true;true;true;true;true;true;true;true;true;true;true;true;true;true;true;true;true;true;true;true;true;true;true;true;true;true;true;true;true;true;true;true;true;true;true;true;true;true;true;true;true;true;true;true;true;true;true;true;true;true;true;true;true;true;true;true;true;true;true;true;true;true;true;true;true;true;true;true;true;true;true;true;true;true;true;true;true;true;true;true;true;true;true;true;true;true;true;true;true;true;true;true;true;true;true;true;true;true;true;true;true;true;true;true;true;true;true;true;true;true;true;true;true;true;true;true;true;true;true;true;true;true;true;true;true;true;true;true;true;true;true;true;true;true;true;true;true;true;true;true;true;true;true;true;true;true;true;true;true;true;true;true;true;true;true;true;true;true;true;true;true;true;true;true;true;true;true;true;true;true;true;true;true;true;true;true;true;true;true;true;true;true;true;true;true;true;true;true;true;true;true;true;true;true;true;true;true;true;true;true;true;true;true;true;true;true;true;true;true;true;true;true;true;true;true;true;true;true;true;true;true;true;true;true;true;true;true;true;true;true;true;true;true;true;true;true;true;true;true;true;true;true;true;true;true;true;true;true;true;true;true;true;true;true;true;true;true;true;true;true;true;true;true;true;true;true;true;true;true;true;true;true;true;true;true;true;true;true;true;true;true;true;true;true;true;true;true;true;true;true;true;true;true;true;true;true;true;true;true;true;true;true;true;true;true;true;true;true;true;true;true;true;true;true;true;true;true;true;true;true;true;true;true;true;true;true;true;true;true;true;true;true;true;true;true;true;true;true;true;true;true;true;true;true;true;true;true;true;true;true;true;true;true;true;true;true;true;true;true;true;true;true;true;true;true;true;true;true;true;true;true;true;true;true;true;true;true;true;true;true;true;true;true;true;true;true;true;true;true;true;true;true;true;true;true;true;true;true;true;true;true;true;true;true;true;true;true;true;true;true;true;true;true;true;true;true;true;true;true;true;true;true;true;true;true;true;true;true;true;true;true;true;true;true;true;true;true;true;true;true;true;true;true;true;true;true;true;true;true;true;true;true;true;true;true;true;true;true;true;true;true;true;true;true;true;true;true;true;true;true;true;true;true;true;true;true;true;true;true;true;true;true;true;true;true;true;true;true;true;true;true;true;true;true;true;true;true;true;true;true;true;true;true;true;true;true;true;true;true;true;true;true;true;true;true;true;true;true;true;true;true;true;true;true;true;true;true;true;true;true;true;true;true;true;true;true;true;true;true;true;true;true;true;true;true;true;true;true;true;true;true;true;true;true;true;true;true;true;true;true;true;true;true;true;true;true;true;true;true;true;true;true;true;true;true;true;true;true;true;true;true;true;true;true;true;true;true;true;true;true;true;true;true;true;true;true;true;true;true;true;true;true;true;true;true;true;true;true;true;true;true;true;true;true;true;true;true;true;true;true;true;true;true;true;true;true;true;true;true;true;true;true;true;true;true;true;true;true;true;true;true;true;true;true;true;true;true;true;true;true;true;true;true;true;true;true;true;true;true;true;true;true;true;true;true;true;true;true;true;true;true;true;true;true;true;true;true;true;true;true;true;true;true;true;true;true;true;true;true;true;true;true;true;true;true;true;true;true;true;true;true;true;true;true;true;true;true;true;true;true;true;true;true;true;true;true;true;true;true;true;true;true;true;true;true;true;true;true;true;true;true;true;true;true;true;true;true;true;true;true;true;true;true;true;true;true;true;true;true;true;true;true;true;true;true;true;true;true;true;true;true;true;true;true;true;true;true;true;true;true;true;true;true;true;true;true;true;true;true;true;true;true;true;true;true;true;true;true;true;true;true;true;true;true;true;true;true;true;true;true;true;true;true;true;true;true;true;true;true;true;true;true;true;true;true;true;true;true;true;true;true;true;true;true;true;true;true;true;true;true;true;true;true;true;true;true;true;true;true;true;true;true;true;true;true;true;true;true;true;true;true;true;true;true;true;true;true;true;true;true;true;true;true;true;true;true;true;true;true;true;true;true;true;true;true;true;true;true;true;true;true;true;true;true;true;true;true;true;true;true;true;true;true;true;true;true;true;true;true;true;true;true;true;true;true;true;true;true;true;true;true;true;true;true;true;true;true;true;true;true;true;true;true;true;true;true;true;true;true;true;true;true;true;true;true;true;true;true;true;true;true;true;true;true;true;true;true;true;true;true;true;true;true;true;true;true;true;true;true;true;true;true;true;true;true;true;true;true;true;true;true;true;true;true;true;true;true;true;true;true;true;true;true;true;true;true;true;true;true;true;true;true;true;true;true;true;true;true;true;true;true;true;true;true;true;true;true;true;true;true;true;true;true;true;true;true;true;true;true;true;true;true;true;true;true;true;true;true;true;true;true;true;true;true;true;true;true;true;true;true;true;true;true;true;true;true;true;true;true;true;true;true;true;true;true;true;true;true;true;true;true;true;true;true;true;true;true;true;true;true;true;true;true;true;true;true;true;true;true;true;true;true;true;true;true;true;true;true;true;true;true;true;true;true;true;true;true;true;true;true;true;true;true;true;true;true;true;true;true;true;true;true;true;true;true;true;true;true;true;true;true;true;true;true;true;true;true;true;true;true;true;true;true;true;true;true;true;true;true;true;true;true;true;true;true;true;true;true;true;true;true;true;true;true;true;true;true;true;true;true;true;true;true;true;true;true;true;true;true;true;true;true;true;true;true;true;true;true;true;true;true;true;true;true;true;true;true;true;true;true;true;true;true;true;true;true;true;true;true;true;true;true;true;true;true;true;true;true;true;true;true;true;true;true;true;true;true;true;true;true;true;true;true;true;true;true;true;true;true;true;true;true;true;true;true;true;true;true;true;true;true;true;true;true;true;true;true;true;true;true;true;true;true;true;true;true;true;true;true;true;true;true;true;true;true;true;true;true;true;true;true;true;true;true;true;true;true;true;true;true;true;true;true;true;true;true;true;true;true;true;true;true;true;true;true;true;true;true;true;true;true;true;true;true;true;true;true;true;true;true;true;true;true;true;true;true;true;true;true;true;true;true;true;true;true;true;true;true;true;true;true;true;true;true;true;true;true;true;true;true;true;true;true;true;true;true;true;true;true;true;true;true;true;true;true;true;true;true;true;true;true;true;true;true;true;true;true;true;true;true;true;true;true;true;true;true;true;true;true;true;true;true;true;true;true;true;true;true;true;true;true;true;true;true;true;true;true;true;true;true;true;true;true;true;true;true;true;true;true;true;true;true;true;true;true;true;true;true;true;true;true;true;true;true;true;true;true;true;true;true;true;true;true;true;true;true;true;true;true;true;true;true;true;true;true;true;true;true;true;true;true;true;true;true;true;true;true;true;true;true;true;true;true;true;true;true;true;true;true;true;true;true;true;true;true;true;true;true;true;true;true;true;true;true;true;true;true;true;true;true;true;true;true;true;true;true;true;true;true;true;true;true;true;true;true;true;true;true;true;true;true;true;true;true;true;true;true;true;true;true;true;true;true;true;true;true;true;true;true;true;true;true;true;true;true;true;true;true;true;true;true;true;true;true;true;true;true;true;true;true;true;true;true;true;true;true;true;true;true;true;true;true;true;true;true;true;true;true;true;true;true;true;true;true;true;true;true;true;true;true;true;true;true;true;true;true;true;true;true;true;true;true;true;true;true;true;true;true;true;true;true;true;true;true;true;true;true;true;true;true;true;true;true;true;true;true;true;true;true;true;true;true;true;true;true;true;true;true;true;true;true;true;true;true;true;true;true;true;true;true;true;true;true;true;true;true;true;true;true;true;true;true;true;true;true;true;true;true;true;true;true;true;true;true;true;true;true;true;true;true;true;true;true;true;true;true;true;true;true;true;true;true;true;true;true;true;true;true;true;true;true;true;true;true;true;true;true;true;true;true;true;true;true;true;true;true;true;true;true;true;true;true;true;true;true;true;true;true;true;true;true;true;true;true;true;true;true;true;true;true;true;true;true;true;true;true;true;true;true;true;true;true;true;true;true;true;true;true;true;true;true;true;true;true;true;true;true;true;true;true;true;true;true;true;true;true;true;true;true;true;true;true;true;true;true;true;true;true;true;true;true;true;true;true;true;true;true;true;true;true;true;true;true;true;true;true;true;true;true;true;true;true;true;true;true;true;true;true;true;true;true;true;true;true;true;true;true;true;true;true;true;true;true;true;true;true;true;true;true;true;true;true;true;true;true;true;true;true;true;true;true;true;true;true;true;true;true;true;true;true;true;true;true;true;true;true;true;true;true;true;true;true;true;true;true;true;true;true;true;true;true;true;true;true;true;true;true;true;true;true;true;true;true;true;true;true;true;true;true;true;true;true;true;true;true;true;true;true;true;true;true;true;true;true;true;true;true;true;true;true;true;true;true;true;true;true;true;true;true;true;true;true;true;true;true;true;true;true;true;true;true;true;true;true;true;true;true;true;true;true;true;true;true;true;true;true;true;true;true;true;true;true;true;true;true;true;true;true;true;true;true;true;true;true;true;true;true;true;true;true;true;true;true;true;true;true;true;true;true;true;true;true;true;true;true;true;true;true;true;true;true;true;true;true;true;true;true;true;true;true;true;true;true;true;true;true;true;true;true;true;true;true;true;true;true;true;true;true;true;true;true;true;true;true;true;true;true;true;true;true;true;true;true;true;true;true;true;true;true;true;true;true;true;true;true;true;true;true;true;true;true;true;true;true;true;true;true;true;true;true;true;true;true;true;true;true;true;true;true;true;true;true;true;true;true;true;true;true;true;true;true;true;true;true;true;true;true;true;true;true;true;true;true;true;true;true;true;true;true;true;true;true;true;true;true;true;true;true;true;true;true;true;true;true;true;true;true;true;true;true;true;true;true;true;true;true;true;true;true;true;true;true;true;true;true;true;true;true;true;true;true;true;true;true;true;true;true;true;true;true;true;true;true;true;true;true;true;true;true;true;true;true;true;true;true;true;true;true;true;true;true;true;true;true;true;true;true;true;true;true;true;true;true;true;true;true;true;true;true;true;true;true;true;true;true;true;true;true;true;true;true;true;true;true;true;true;true;true;true;true;true;true;true;true;true;true;true;true;true;true;true;true;true;true;true;true;true;true;true;true;true;true;true;true;true;true;true;true;true;true;true;true;true;true;true;true;true;true;true;true;true;true;true;true;true;true;true;true;true;true;true;true;true;true;true;true;true;true;true;true;true;true;true;true;true;true;true;true;true;true;true;true;true;true;true;true;true;true;true;true;true;true;true;true;true;true;true;true;true;true;true;true;true;true;true;true;true;true;true;true;true;true;true;true;true;true;true;true;true;true;true;true;true;true;true;true;true;true;true;true;true;true;true;true;true;true;true;true;true;true;true;true;true;true;true;true;true;true;true;true;true;true;true;true;true;true;true;true;true;true;true;true;true;true;true;true;true;true;true;true;true;true;true;true;true;true;true;true;true;true;true;true;true;true;true;true;true;true;true;true;true;true;true;true;true;true;true;true;true;true;true;true;true;true;true;true;true;true;true;true;true;true;true;true;true;true;true;true;true;true;true;true;true;true;true;true;true;true;true;true;true;true;true;true;true;true;true;true;true;true;true;true;true;true;true;true;true;true;true;true;true;true;true;true;true;true;true;true;true;true;true;true;true;true;true;true;true;true;true;true;true;true;true;true;true;true;true;true;true;true;true;true;true;true;true;true;true;true;true;true;true;true;true;true;true;true;true;true;true;true;true;true;true;true;true;true;true;true;true;true;true;true;true;true;true;true;true;true;true;true;true;true;true;true;true;true;true;true;true;true;true;true;true;true;true;true;true;true;true;true;true;true;true;true;true;true;true;true;true;true;true;true;true;true;true;true;true;true;true;true;true;true;true;true;true;true;true;true;true;true;true;true;true;true;true;true;true;true;true;true;true;true;true;true;true;true;true;true;true;true;true;true;true;true;true;true;true;true;true;true;true;true;true;true;true;true;true;true;true;true;true;true;true;true;true;true;true;true;true;true;true;true;true;true;true;true;true;true;true;true;true;true;true;true;true;true;true;true;true;true;true;true;true;true;true;true;true;true;true;true;true;true;true;true;true;true;true;true;true;true;true;true;true;true;true;true;true;true;true;true;true;true;true;true;true;true;true;true;true;true;true;true;true;true;true;true;true;true;true;true;true;true;true;true;true;true;true;true;true;true;true;true;true;true;true;true;true;true;true;true;true;true;true;true;true;true;true;true;true;true;true;true;true;true;true;true;true;true;true;true;true;true;true;true;true;true;true;true;true;true;true;true;true;true;true;true;true;true;true;true;true;true;true;true;true;true;true;true;true;true;true;true;true;true;true;true;true;true;true;true;true;true;true;true;true;true;true;true;true;true;true;true;true;true;true;true;true;true;true;true;true;true;true;true;true;true;true;true;true;true;true;true;true;true;true;true;true;true;true;true;true;true;true;true;true;true;true;true;true;true;true;true;true;true;true;true;true;true;true;true;true;true;true;true;true;true;true;true;true;true;true;true;true;true;true;true;true;true;true;true;true;true;true;true;true;true;true;true;true;true;true;true;true;true;true;true;true;true;true;true;true;true;true;true;true;true;true;true;true;true;true;true;true;true;true;true;true;true;true;true;true;true;true;true;true;true;true;true;true;true;true;true;true;true;true;true;true;true;true;true;true;true;true;true;true;true;true;true;true;true;true;true;true;true;true;true;true;true;true;true;true;true;true;true;true;true;true;true;true;true;true;true;true;true;true;true;true;true;true;true;true;true;true;true;true;true;true;true;true;true;true;true;true;true;true;true;true;true;true;true;true;true;true;true;true;true;true;true;true;true;true;true;true;true;true;true;true;true;true;true;true;true;true;true;true;true;true;true;true;true;true;true;true;true;true;true;true;true;true;true;true;true;true;true;true;true;true;true;true;true;true;true;true;true;true;true;true;true;true;true;true;true;true;true;true;true;true;true;true;true;true;true;true;true;true;true;true;true;true;true;true;true;true;true;true;true;true;true;true;true;true;true;true;true;true;true;true;true;true;true;true;true;true;true;true;true;true;true;true;true;true;true;true;true;true;true;true;true;true;true;true;true;true;true;true;true;true;true;true;true;true;true;true;true;true;true;true;true;true;true;true;true;true;true;true;true;true;true;true;true;true;true;true;true;true;true;true;true;true;true;true;true;true;true;true;true;true;true;true;true;true;true;true;true;true;true;true;true;true;true;true;true;true;true;true;true;true;true;true;true;true;true;true;true;true;true;true;true;true;true;true;true;true;true;true;true;true;true;true;true;true;true;true;true;true;true;true;true;true;true;true;true;true;true;true;true;true;true;true;true;true;true;true;true;true;true;true;true;true;true;true;true;true;true;true;true;true;true;true;true;true;true;true;true;true;true;true;true;true;true;true;true;true;true;true;true;true;true;true;true;true;true;true;true;true;true;true;true;true;true;true;true;true;true;true;true;true;true;true;true;true;true;true;true;true;true;true;true;true;true;true;true;true;true;true;true;true;true;true;true;true;true;true;true;true;true;true;true;true;true;true;true;true;true;true;true;true;true;true;true;true;true;true;true;true;true;true;true;true;true;true;true;true;true;true;true;true;true;true;true;true;true;true;true;true;true;true;true;true;true;true;true;true;true;true;true;true;true;true;true;true;true;true;true;true;true;true;true;true;true;true;true;true;true;true;true;true;true;true;true;true;true;true;true;true;true;true;true;true;true;true;true;true;true;true;true;true;true;true;true;true;true;true;true;true;true;true;true;true;true;true;true;true;true;true;true;true;true;true;true;true;true;true;true;true;true;true;true;true;true;true;true;true;true;true;true;true;true;true;true;true;true;true;true;true;true;true;true;true;true;true;true;true;true;true;true;true;true;true;true;true;true;true;true;true;true;true;true;true;true;true;true;true;true;true;true;true;true;true;true;true;true;true;true;true;true;true;true;true;true;true;true;true;true;true;true;true;true;true;true;true;true;true;true;true;true;true;true;true;true;true;true;true;true;true;true;true;true;true;true;true;true;true;true;true;true;true;true;true;true;true;true;true;true;true;true;true;true;true;true;true;true;true;true;true;true;true;true;true;true;true;true;true;true;true;true;true;true;true;true;true;true;true;true;true;true;true;true;true;true;true;true;true;true;true;true;true;true;true;true;true;true;true;true;true;true;true;true;true;true;true;true;true;true;true;true;true;true;true;true;true;true;true;true;true;true;true;true;true;true;true;true;true;true;true;true;true;true;true;true;true;true;true;true;true;true;true;true;true;true;true;true;true;true;true;true;true;true;true;true;true;true;true;true;true;true;true;true;true;true;true;true;true;true;true;true;true;true;true;true;true;true;true;true;true;true;true;true;true;true;true;true;true;true;true;true;true;true;true;true;true;true;true;true;true;true;true;true;true;true;true;true;true;true;true;true;true;true;true;true;true;true;true;true;true;true;true;true;true;true;true;true;true;true;true;true;true;true;true;true;true;true;true;true;true;true;true;true;true;true;true;true;true;true;true;true;true;true;true;true;true;true;true;true;true;true;true;true;true;true;true;true;true;true;true;true;true;true;true;true;true;true;true;true;true;true;true;true;true;true;true;true;true;true;true;true;true;true;true;true;true;true;true;true;true;true;true;true;true;true;true;true;true;true;true;true;true;true;true;true;true;true;true;true;true;true;true;true;true;true;true;true;true;true;true;true;true;true;true;true;true;true;true;true;true;true;true;true;true;true;true;true;true;true;true;true;true;true;true;true;true;true;true;true;true;true;true;true;true;true;true;true;true;true;true;true;true;true;true;true;true;true;true;true;true;true;true;true;true;true;true;true;true;true;true;true;true;true;true;true;true;true;true;true;true;true;true;true;true;true;true;true;true;true;true;true;true;true;true;true;true;true;true;true;true;true;true;true;true;true;true;true;true;true;true;true;true;true;true;true;true;true;true;true;true;true;true;true;true;true;true;true;true;true;true;true;true;true;true;true;true;true;true;true;true;true;true;true;true;true;true;true;true;true;true;true;true;true;true;true;true;true;true;true;true;true;true;true;true;true;true;true;true;true;true;true;true;true;true;true;true;true;true;true;true;true;true;true;true;true;true;true;true;true;true;true;true;true;true;true;true;true;true;true;true;true;true;true;true;true;true;true;true;true;true;true;true;true;true;true;true;true;true;true;true;true;true;true;true;true;true;true;true;true;true;true;true;true;true;true;true;true;true;true;true;true;true;true;true;true;true;true;true;true;true;true;true;true;true;true;true;true;true;true;true;true;true;true;true;true;true;true;true;true;true;true;true;true;true;true;true;true;true;true;true;true;true;true;true;true;true;true;true;true;true;true;true;true;true;true;true;true;true;true;true;true;true;true;true;true;true;true;true;true;true;true;true;true;true;true;true;true;true;true;true;true;true;true;true;true;true;true;true;true;true;true;true;true;true;true;true;true;true;true;true;true;true;true;true;true;true;true;true;true;true;true;true;true;true;true;true;true;true;true;true;true;true;true;true;true;true;true;true;true;true;true;true;true;true;true;true;true;true;true;true;true;true;true;true;true;true;true;true;true;true;true;true;true;true;true;true;true;true;true;true;true;true;true;true;true;true;true;true;true;true;true;true;true;true;true;true;true;true;true;true;true;true;true;true;true;true;true;true;true;true;true;true;true;true;true;true;true;true;true;true;true;true;true;true;true;true;true;true;true;true;true;true;true;true;true;true;true;true;true;true;true;true;true;true;true;true;true;true;true;true;true;true;true;true;true;true;true;true;true;true;true;true;true;true;true;true;true;true;true;true;true;true;true;true;true;true;true;true;true;true;true;true;true;true;true;true;true;true;true;true;true;true;true;true;true;true;true;true;true;true;true;true;true;true;true;true;true;true;true;true;true;true;true;true;true;true;true;true;true;true;true;true;true;true;true;true;true;true;true;true;true;true;true;true;true;true;true;true;true;true;true;true;true;true;true;true;true;true;true;true;true;true;true;true;true;true;true;true;true;true;true;true;true;true;true;true;true;true;true;true;true;true;true;true;true;true;true;true;true;true;true;true;true;true;true;true;true;true;true;true;true;true;true;true;true;true;true;true;true;true;true;true;true;true;true;true;true;true;true;true;true;true;true;true;true;true;true;true;true;true;true;true;true;true;true;true;true;true;true;true;true;true;true;true;true;true;true;true;true;true;true;true;true;true;true;true;true;true;true;true;true;true;true;true;true;true;true;true;true;true;true;true;true;true;true;true;true;true;true;true;true;true;true;true;true;true;true;true;true;true;true;true;true;true;true;true;true;true;true;true;true;true;true;true;true;true;true;true;true;true;true;true;true;true;true;true;true;true;true;true;true;true;true;true;true;true;true;true;true;true;true;true;true;true;true;true;true;true;true;true;true;true;true;true;true;true;true;true;true;true;true;true;true;true;true;true;true;true;true;true;true;true;true;true;true;true;true;true;true;true;true;true;true;true;true;true;true;true;true;true;true;true;true;true;true;true;true;true;true;true;true;true;true;true;true;true;true;true;true;true;true;true;true;true;true;true;true;true;true;true;true;true;true;true;true;true;true;true;true;true;true;true;true;true;true;true;true;true;true;true;true;true;true;true;true;true;true;true;true;true;true;true;true;true;true;true;true;true;true;true;true;true;true;true;true;true;true;true;true;true;true;true;true;true;true;true;true;true;true;true;true;true;true;true;true;true;true;true;true;true;true;true;true;true;true;true;true;true;true;true;true;true;true;true;true;true;true;true;true;true;true;true;true;true;true;true;true;true;true;true;true;true;true;true;true;true;true;true;true;true;true;true;true;true;true;true;true;true;true;true;true;true;true;true;true;true;true;true;true;true;true;true;true;true;true;true;true;true;true;true;true;true;true;true;true;true;true;true;true;true;true;true;true;true;true;true;true;true;true;true;true;true;true;true;true;true;true;true;true;true;true;true;true;true;true;true;true;true;true;true;true;true;true;true;true;true;true;true;true;true;true;true;true;true;true;true;true;true;true;true;true;true;true;true;true;true;true;true;true;true;true;true;true;true;true;true;true;true;true;true;true;true;true;true;true;true;true;true;true;true;true;true;true;true;true;true;true;true;true;true;true;true;true;true;true;true;true;true;true;true;true;true;true;true;true;true;true;true;true;true;true;true;true;true;true;true;true;true;true;true;true;true;true;true;true;true;true;true;true;true;true;true;true;true;true;true;true;true;true;true;true;true;true;true;true;true;true;true;true;true;true;true;true;true;true;true;true;true;true;true;true;true;true;true;true;true;true;true;true;true;true;true;true;true;true;true;true;true;true;true;true;true;true;true;true;true;true;true;true;true;true;true;true;true;true;true;true;true;true;true;true;true;true;true;true;true;true;true;true;true;true;true;true;true;true;true;true;true;true;true;true;true;true;true;true;true;true;true;true;true;true;true;true;true;true;true;true;true;true;true;true;true;true;true;true;true;true;true;true;true;true;true;true;true;true;true;true;true;true;true;true;true;true;true;true;true;true;true;true;true;true;true;true;true;true;true;true;true;true;true;true;true;true;true;true;true;true;true;true;true;true;true;true;true;true;true;true;true;true;true;true;true;true;true;true;true;true;true;true;true;true;true;true;true;true;true;true;true;true;true;true;true;true;true;true;true;true;true;true;true;true;true;true;true;true;true;true;true;true;true;true;true;true;true;true;true;true;true;true;true;true;true;true;true;true;true;true;true;true;true;true;true;true;true;true;true;true;true;true;true;true;true;true;true;true;true;true;true;true;true;true;true;true;true;true;true;true;true;true;true;true;true;true;true;true;true;true;true;true;true;true;true;true;true;true;true;true;true;true;true;true;true;true;true;true;true;true;true;true;true;true;true;true;true;true;true;true;true;true;true;true;true;true;true;true;true;true;true;true;true;true;true;true;true;true;true;true;true;true;true;true;true;true;true;true;true;true;true;true;true;true;true;true;true;true;true;true;true;true;true;true;true;true;true;true;true;true;true;true;true;true;true;true;true;true;true;true;true;true;true;true;true;true;true;true;true;true;true;true;true;true;true;true;true;true;true;true;true;true;true;true;true;true;true;true;true;true;true;true;true;true;true;true;true;true;true;true;true;true;true;true;true;true;true;true;true;true;true;true;true;true;true;true;true;true;true;true;true;true;true;true;true;true;true;true;true;true;true;true;true;true;true;true;true;true;true;true;true;true;true;true;true;true;true;true;true;true;true;true;true;true;true;true;true;true;true;true;true;true;true;true;true;true;true;true;true;true;true;true;true;true;true;true;true;true;true;true;true;true;true;true;true;true;true;true;true;true;true;true;true;true;true;true;true;true;true;true;true;true;true;true;true;true;true;true;true;true;true;true;true;true;true;true;true;true;true;true;true;true;true;true;true;true;true;true;true;true;true;true;true;true;true;true;true;true;true;true;true;true;true;true;true;true;true;true;true;true;true;true;true;true;true;true;true;true;true;true;true;true;true;true;true;true;true;true;true;true;true;true;true;true;true;true;true;true;true;true;true;true;true;true;true;true;true;true;true;true;true;true;true;true;true;true;true;true;true;true;true;true;true;true;true;true;true;true;true;true;true;true;true;true;true;true;true;true;true;true;true;true;true;true;true;true;true;true;true;true;true;true;true;true;true;true;true;true;true;true;true;true;true;true;true;true;true;true;true;true;true;true;true;true;true;true;true;true;true;true;true;true;true;true;true;true;true;true;true;true;true;true;true;true;true;true;true;true;true;true;true;true;true;true;true;true;true;true;true;true;true;true;true;true;true;true;true;true;true;true;true;true;true;true;true;true;true;true;true;true;true;true;true;true;true;true;true;true;true;true;true;true;true;true;true;true;true;true;true;true;true;true;true;true;true;true;true;true;true;true;true;true;true;true;true;true;true;true;true;true;true;true;true;true;true;true;true;true;true;true;true;true;true;true;true;true;true;true;true;true;true;true;true;true;true;true;true;true;true;true;true;true;true;true;true;true;true;true;true;true;true;true;true;true;true;true;true;true;true;true;true;true;true;true;true;true;true;true;true;true;true;true;true;true;true;true;true;true;true;true;true;true;true;true;true;true;true;true;true;true;true;true;true;true;true;true;true;true;true;true;true;true;true;true;true;true;true;true;true;true;true;true;true;true;true;true;true;true;true;true;true;true;true;true;true;true;true;true;true;true;true;true;true;true;true;true;true;true;true;true;true;true;true;true;true;true;true;true;true;true;true;true;true;true;true;true;true;true;true;true;true;true;true;true;true;true;true;true;true;true;true;true;true;true;true;true;true;true;true;true;true;true;true;true;true;true;true;true;true;true;true;true;true;true;true;true;true;true;true;true;true;true;true;true;true;true;true;true;true;true;true;true;true;true;true;true;true;true;true;true;true;true;true;true;true;true;true;true;true;true;true;true;true;true;true;true;true;true;true;true;true;true;true;true;true;true;true;true;true;true;true;true;true;true;true;true;true;true;true;true;true;true;true;true;true;true;true;true;true;true;true;true;true;true;true;true;true;true;true;true;true;true;true;true;true;true;true;true;true;true;true;true;true;true;true;true;true;true;true;true;true;true;true;true;true;true;true;true;true;true;true;true;true;true;true;true;true;true;true;true;true;true;true;true;true;true;true;true;true;true;true;true;true;true;true;true;true;true;true;true;true;true;true;true;true;true;true;true;true;true;true;true;true;true;true;true;true;true;true;true;true;true;true;true;true;true;true;true;true;true;true;true;true;true;true;true;true;true;true;true;true;true;true;true;true;true;true;true;true;true;true;true;true;true;true;true;true;true;true;true;true;true;true;true;true;true;true;true;true;true;true;true;true;true;true;true;true;true;true;true;true;true;true;true;true;true;true;true;true;true;true;true;true;true;true;true;true;true;true;true;true;true;true;true;true;true;true;true;true;true;true;true;true;true;true;true;true;true;true;true;true;true;true;true;true;true;true;true;true;true;true;true;true;true;true;true;true;true;true;true;true;true;true;true;true;true;true;true;true;true;true;true;true;true;true;true;true;true;true;true;true;true;true;true;true;true;true;true;true;true;true;true;true;true;true;true;true;true;true;true;true;true;true;true;true;true;true;true;true;true;true;true;true;true;true;true;true;true;true;true;true;true;true;true;true;true;true;true;true;true;true;true;true;true;true;true;true;true;true;true;true;true;true;true;true;true;true;true;true;true;true;true;true;true;true;true;true;true;true;true;true;true;true;true;true;true;true;true;true;true;true;true;true;true;true;true;true;true;true;true;true;true;true;true;true;true;true;true;true;true;true;true;true;true;true;true;true;true;true;true;true;true;true;true;true;true;true;true;true;true;true;true;true;true;true;true;true;true;true;true;true;true;true;true;true;true;true;true;true;true;true;true;true;true;true;true;true;true;true;true;true;true;true;true;true;true;true;true;true;true;true;true;true;true;true;true;true;true;true;true;true;true;true;true;true;true;true;true;true;true;true;true;true;true;true;true;true;true;true;true;true;true;true;true;true;true;true;true;true;true;true;true;true;true;true;true;true;true;true;true;true;true;true;true;true;true;true;true;true;true;true;true;true;true;true;true;true;true;true;true;true;true;true;true;true;true;true;true;true;true;true;true;true;true;true;true;true;true;true;true;true;true;true;true;true;true;true;true;true;true;true;true;true;true;true;true;true;true;true;true;true;true;true;true;true;true;true;true;true;true;true;true;true;true;true;true;true;true;true;true;true;true;true;true;true;true;true;true;true;true;true;true;true;true;true;true;true;true;true;true;true;true;true;true;true;true;true;true;true;true;true;true;true;true;true;true;true;true;true;true;true;true;true;true;true;true;true;true;true;true;true;true;true;true;true;true;true;true;true;true;true;true;true;true;true;true;true;true;true;true;true;true;true;true;true;true;true;true;true;true;true;true;true;true;true;true;true;true;true;true;true;true;true;true;true;true;true;true;true;true;true;true;true;true;true;true;true;true;true;true;true;true;true;true;true;true;true;true;true;true;true;true;true;true;true;true;true;true;true;true;true;true;true;true;true;true;true;true;true;true;true;true;true;true;true;true;true;true;true;true;true;true;true;true;true;true;true;true;true;true;true;true;true;true;true;true;true;true;true;true;true;true;true;true;true;true;true;true;true;true;true;true;true;true;true;true;true;true;true;true;true;true;true;true;true;true;true;true;true;true;true;true;true;true;true;true;true;true;true;true;true;true;true;true;true;true;true;true;true;true;true;true;true;true;true;true;true;true;true;true;true;true;true;true;true;true;true;true;true;true;true;true;true;true;true;true;true;true;true;true;true;true;true;true;true;true;true;true;true;true;true;true;true;true;true;true;true;true;true;true;true;true;true;true;true;true;true;true;true;true;true;true;true;true;true;true;true;true;true;true;true;true;true;true;true;true;true;true;true;true;true;true;true;true;true;true;true;true;true;true;true;true;true;true;true;true;true;true;true;true;true;true;true;true;true;true;true;true;true;true;true;true;true;true;true;true;true;true;true;true;true;true;true;true;true;true;true;true;true;true;true;true;true;true;true;true;true;true;true;true;true;true;true;true;true;true;true;true;true;true;true;true;true;true;true;true;true;true;true;true;true;true;true;true;true;true;true;true;true;true;true;true;true;true;true;true;true;true;true;true;true;true;true;true;true;true;true;true;true;true;true;true;true;true;true;true;true;true;true;true;true;true;true;true;true;true;true;true;true;true;true;true;true;true;true;true;true;true;true;true;true;true;true;true;true;true;true;true;true;true;true;true;true;true;true;true;true;true;true;true;true;true;true;true;true;true;true;true;true;true;true;true;true;true;true;true;true;true;true;true;true;true;true;true;true;true;true;true;true;true;true;true;true;true;true;true;true;true;true;true;true;true;true;true;true;true;true;true;true;true;true;true;true;true;true;true;true;true;true;true;true;true;true;true;true;true;true;true;true;true;true;true;true;true;true;true;true;true;true;true;true;true;true;true;true;true;true;true;true;true;true;true;true;true;true;true;true;true;true;true;true;true;true;true;true;true;true;true;true;true;true;true;true;true;true;true;true;true;true;true;true;true;true;true;true;true;true;true;true;true;true;true;true;true;true;true;true;true;true;true;true;true;true;true;true;true;true;true;true;true;true;true;true;true;true;true;true;true;true;true;true;true;true;true;true;true;true;true;true;true;true;true;true;true;true;true;true;true;true;true;true;true;true;true;true;true;true;true;true;true;true;true;true;true;true;true;true;true;true;true;true;true;true;true;true;true;true;true;true;true;true;true;true;true;true;true;true;true;true;true;true;true;true;true;true;true;true;true;true;true;true;true;true;true;true;true;true;true;true;true;true;true;true;true;true;true;true;true;true;true;true;true;true;true;true;true;true;true;true;true;true;true;true;true;true;true;true;true;true;true;true;true;true;true;true;true;true;true;true;true;true;true;true;true;true;true;true;true;true;true;true;true;true;true;true;true;true;true;true;true;true;true;true;true;true;true;true;true;true;true;true;true;true;true;true;true;true;true;true;true;true;true;true;true;true;true;true;true;true;true;true;true;true;true;true;true;true;true;true;true;true;true;true;true;true;true;true;true;true;true;true;true;true;true;true;true;true;true;true;true;true;true;true;true;true;true;true;true;true;true;true;true;true;true;true;true;true;true;true;true;true;true;true;true;true;true;true;true;true;true;true;true;true;true;true;true;true;true;true;true;true;true;true;true;true;true;true;true;true;true;true;true;true;true;true;true;true;true;true;true;true;true;true;true;true;true;true;true;true;true;true;true;true;true;true;true;true;true;true;true;true;true;true;true;true;true;true;true;true;true;true;true;true;true;true;true;true;true;true;true;true;true;true;true;true;true;true;true;true;true;true;true;true;true;true;true;true;true;true;true;true;true;true;true;true;true;true;true;true;true;true;true;true;true;true;true;true;true;true;true;true;true;true;true;true;true;true;true;true;true;true;true;true;true;true;true;true;true;true;true;true;true;true;true;true;true;true;true;true;true;true;true;true;true;true;true;true;true;true;true;true;true;true;true;true;true;true;true;true;true;true;true;true;true;true;true;true;true;true;true;true;true;true;true;true;true;true;true;true;true;true;true;true;true;true;true;true;true;true;true;true;true;true;true;true;true;true;true;true;true;true;true;true;true;true;true;true;true;true;true;true;true;true;true;true;true;true;true;true;true;true;true;true;true;true;true;true;true;true;true;true;true;true;true;true;true;true;true;true;true;true;true;true;true;true;true;true;true;true;true;true;true;true;true;true;true;true;true;true;true;true;true;true;true;true;true;true;true;true;true;true;true;true;true;true;true;true;true;true;true;true;true;true;true;true;true;true;true;true;true;true;true;true;true;true;true;true;true;true;true;true;true;true;true;true;true;true;true;true;true;true;true;true;true;true;true;true;true;true;true;true;true;true;true;true;true;true;true;true;true;true;true;true;true;true;true;true;true;true;true;true;true;true;true;true;true;true;true;true;true;true;true;true;true;true;true;true;true;true;true;true;true;true;true;true;true;true;true;true;true;true;true;true;true;true;true;true;true;true;true;true;true;true;true;true;true;true;true;true;true;true;true;true;true;true;true;true;true;true;true;true;true;true;true;true;true;true;true;true;true;true;true;true;true;true;true;true;true;true;true;true;true;true;true;true;true;true;true;true;true;true;true;true;true;true;true;true;true;true;true;true;true;true;true;true;true;true;true;true;true;true;true;true;true;true;true;true;true;true;true;true;true;true;true;true;true;true;true;true;true;true;true;true;true;true;true;true;true;true;true;true;true;true;true;true;true;true;true;true;true;true;true;true;true;true;true;true;true;true;true;true;true;true;true;true;true;true;true;true;true;true;true;true;true;true;true;true;true;true;true;true;true;true;true;true;true;true;true;true;true;true;true;true;true;true;true;true;true;true;true;true;true;true;true;true;true;true;true;true;true;true;true;true;true;true;true;true;true;true;true;true;true;true;true;true;true;true;true;true;true;true;true;true;true;true;true;true;true;true;true;true;true;true;true;true;true;true;true;true;true;true;true;true;true;true;true;true;true;true;true;true;true;true;true;true;true;true;true;true;true;true;true;true;true;true;true;true;true;true;true;true;true;true;true;true;true;true;true;true;true;true;true;true;true;true;true;true;true;true;true;true;true;true;true;true;true;true;true;true;true;true;true;true;true;true;true;true;true;true;true;true;true;true;true;true;true;true;true;true;true;true;true;true;true;true;true;true;true;true;true;true;true;true;true;true;true;true;true;true;true;true;true;true;true;true;true;true;true;true;true;true;true;true;true;true;true;true;true;true;true;true;true;true;true;true;true;true;true;true;true;true;true;true;true;true;true;true;true;true;true;true;true;true;true;true;true;true;true;true;true;true;true;true;true;true;true;true;true;true;true;true;true;true;true;true;true;true;true;true;true;true;true;true;true;true;true;true;true;true;true;true;true;true;true;true;true;true;true;true;true;true;true;true;true;true;true;true;true;true;true;true;true;true;true;true;true;true;true;true;true;true;true;true;true;true;true;true;true;true;true;true;true;true;true;true;true;true;true;true;true;true;true;true;true;true;true;true;true;true;true;true;true;true;true;true;true;true;true;true;true;true;true;true;true;true;true;true;true;true;true;true;true;true;true;true;true;true;true;true;true;true;true;true;true;true;true;true;true;true;true;true;true;true;true;true;true;true;true;true;true;true;true;true;true;true;true;true;true;true;true;true;true;true;true;true;true;true;true;true;true;true;true;true;true;true;true;true;true;true;true;true;true;true;true;true;true;true;true;true;true;true;true;true;true;true;true;true;true;true;true;true;true;true;true;true;true;true;true;true;true;true;true;true;true;true;true;true;true;true;true;true;true;true;true;true;true;true;true;true;true;true;true;true;true;true;true;true;true;true;true;true;true;true;true;true;true;true;true;true;true;true;true;true;true;true;true;true;true;true;true;true;true;true;true;true;true;true;true;true;true;true;true;true;true;true;true;true;true;true;true;true;true;true;true;true;true;true;true;true;true;true;true;true;true;true;true;true;true;true;true;true;true;true;true;true;true;true;true;true;true;true;true;true;true;true;true;true;true;true;true;true;true;true;true;true;true;true;true;true;true;true;true;true;true;true;true;true;true;true;true;true;true;true;true;true;true;true;true;true;true;true;true;true;true;true;true;true;true;true;true;true;true;true;true;true;true;true;true;true;true;true;true;true;true;true;true;true;true;true;true;true;true;true;true;true;true;true;true;true;true;true;true;true;true;true;true;true;true;true;true;true;true;true;true;true;true;true;true;true;true;true;true;true;true;true;true;true;true;true;true;true;true;true;true;true;true;true;true;true;true;true;true;true;true;true;true;true;true;true;true;true;true;true;true;true;true;true;true;true;true;true;true;true;true;true;true;true;true;true;true;true;true;true;true;true;true;true;true;true;true;true;true;true;true;true;true;true;true;true;true;true;true;true;true;true;true;true;true;true;true;true;true;true;true;true;true;true;true;true;true;true;true;true;true;true;true;true;true;true;true;true;true;true;true;true;true;true;true;true;true;true;true;true;true;true;true;true;true;true;true;true;true;true;true;true;true;true;true;true;true;true;true;true;true;true;true;true;true;true;true;true;true;true;true;true;true;true;true;true;true;true;true;true;true;true;true;true;true;true;true;true;true;true;true;true;true;true;true;true;true;true;true;true;true;true;true;true;true;true;true;true;true;true;true;true;true;true;true;true;true;true;true;true;true;true;true;true;true;true;true;true;true;true;true;true;true;true;true;true;true;true;true;true;true;true;true;true;true;true;true;true;true;true;true;true;true;true;true;true;true;true;true;true;true;true;true;true;true;true;true;true;true;true;true;true;true;true;true;true;true;true;true;true;true;true;true;true;true;true;true;true;true;true;true;true;true;true;true;true;true;true;true;true;true;true;true;true;true;true;true;true;true;true;true;true;true;true;true;true;true;true;true;true;